simulink model "TIM_5_1_2"  (R2022b)
(part 3 of 4)

  Wire_16a (50) : M-S-Function  FunctionName=cisia_msfun  Parameters=Parameter1, Parameter2, Parameter3, resources, Parameter10, codeupdate, step_received, step_computed, dynamic_computed, step_sended, id_entity, id_project, id_type, name_type, color  mask(S-function:msfcn_unit_delay){Parameter1='Wire_16a', Parameter2=1, Parameter3='ORO', resources=|, Parameter10=off, codeupdate=off, step_received=|, step_computed=, dynamic_computed=, step_sended=|, id_entity=50, id_project=38, id_type=1, name_type=Optical_Wire, color=#99CCFF}
      mask resources=|
      | *** INPUT RESOURCES ***
      | NUM_INPUTS 4
      | TLC_CONN (20)
      | TLC_SERVICE (20)
      | CYBER_FAULT (10)
      | MECH_FAULT (1)
      |
      | *** STATE VARIABLES ***
      | NUM_VARIABLES 11
      | Operative_Level(NUMERIC)(1)(1)
      | TLC_services(NUMERIC_ARRAY)(20)(0  0  0  0  0  0  0  0  0  0  0  0  0  0  0  0  0  0  0  0)
      | Connection(NUMERIC_ARRAY)(20)(0  0  0  0  0  0  0  0  0  0  0  0  0  0  0  0  0  0  0  0)
      | Dos_attack(NUMERIC)(1)(0)
      | MITM_attack(NUMERIC)(1)(0)
      | Virus_Attack(NUMERIC)(1)(0)
      | Port_Scan_Attack(NUMERIC)(1)(0)
      | Cyber_Fault(NUMERIC_ARRAY)(10)(0  0  0  0  0  0  0  0  0  0)
      | Mechanical_Fault(NUMERIC)(1)(0)
      | Conn_Fault(NUMERIC)(1)(0)
      | TLC_revoke(NUMERIC_ARRAY)(20)(0  0  0  0  0  0  0  0  0  0  0  0  0  0  0  0  0  0  0  0)
      |
      | *** OUTPUT RESOURCES ***
      | NUM_OUTPUTS 4
      | TLC_CONN (20)
      | TLC_SERVICE (20)
      | CYBER_FAULT (10)
      | MECH_FAULT (1)
      mask step_received=|
      | Connection=max(Connection_init,TLC_CONN);
      | TLC_services=max(TLC_services_init,TLC_SERVICE);
      | TLC_services=mod(TLC_services,10);
      | TLC_revoke=floor(TLC_SERVICE/10);
      |
      | Cyber_Fault=CYBER_FAULT;
      |
      | Mechanical_Fault=max([Mechanical_Fault MECH_FAULT Mechanical_Fault_init]);
      |
      | %TLC_services=TLC_services.*(1-TLC_revoke);
      |
      | Operative_Level=1-Mechanical_Fault;
      mask step_sended=|
      | TLC_CONN=Connection*Operative_Level;
      | TLC_SERVICE=TLC_services*Operative_Level+TLC_revoke*10;
      |
      |
      | CYBER_FAULT=Cyber_Fault*Operative_Level;
      | MECH_FAULT=Mechanical_Fault;
      mask prompts: Parameter1 "entity name"; Parameter2 "sampling time"; Parameter3 "project"; resources "input resources and state variables"; Parameter10 "Bring state variables to output"; codeupdate "update code from mask"
      mask help: This is a level-2 MATLAB file S-function which demonstrates CISIA entity
      mask DialogControl Container1 Prompt: All parameters
      mask Display: image('Icons/Optical_Wire.png')
  Wire_17 (187) : M-S-Function  FunctionName=cisia_msfun  Parameters=Parameter1, Parameter2, Parameter3, resources, Parameter10, codeupdate, step_received, step_computed, dynamic_computed, step_sended, id_entity, id_project, id_type, name_type, color  mask(S-function:msfcn_unit_delay){Parameter1='Wire_17', Parameter2=1, Parameter3='ORO', resources=|, Parameter10=off, codeupdate=off, step_received=|, step_computed=, dynamic_computed=, step_sended=|, id_entity=187, id_project=38, id_type=1, name_type=Optical_Wire, color=#99CCFF}
      mask resources=|
      | *** INPUT RESOURCES ***
      | NUM_INPUTS 4
      | TLC_CONN (20)
      | TLC_SERVICE (20)
      | CYBER_FAULT (10)
      | MECH_FAULT (1)
      |
      | *** STATE VARIABLES ***
      | NUM_VARIABLES 11
      | Operative_Level(NUMERIC)(1)(1)
      | TLC_services(NUMERIC_ARRAY)(20)(0  0  0  0  0  0  0  0  0  0  0  0  0  0  0  0  0  0  0  0)
      | Connection(NUMERIC_ARRAY)(20)(0  0  0  0  0  0  0  0  0  0  0  0  0  0  0  0  0  0  0  0)
      | Dos_attack(NUMERIC)(1)(0)
      | MITM_attack(NUMERIC)(1)(0)
      | Virus_Attack(NUMERIC)(1)(0)
      | Port_Scan_Attack(NUMERIC)(1)(0)
      | Cyber_Fault(NUMERIC_ARRAY)(10)(0  0  0  0  0  0  0  0  0  0)
      | Mechanical_Fault(NUMERIC)(1)(0)
      | Conn_Fault(NUMERIC)(1)(0)
      | TLC_revoke(NUMERIC_ARRAY)(20)(0  0  0  0  0  0  0  0  0  0  0  0  0  0  0  0  0  0  0  0)
      |
      | *** OUTPUT RESOURCES ***
      | NUM_OUTPUTS 4
      | TLC_CONN (20)
      | TLC_SERVICE (20)
      | CYBER_FAULT (10)
      | MECH_FAULT (1)
      mask step_received=|
      | Connection=max(Connection_init,TLC_CONN);
      | TLC_services=max(TLC_services_init,TLC_SERVICE);
      | TLC_services=mod(TLC_services,10);
      | TLC_revoke=floor(TLC_SERVICE/10);
      |
      | Cyber_Fault=CYBER_FAULT;
      |
      | Mechanical_Fault=max([Mechanical_Fault MECH_FAULT Mechanical_Fault_init]);
      |
      | %TLC_services=TLC_services.*(1-TLC_revoke);
      |
      | Operative_Level=1-Mechanical_Fault;
      mask step_sended=|
      | TLC_CONN=Connection*Operative_Level;
      | TLC_SERVICE=TLC_services*Operative_Level+TLC_revoke*10;
      |
      |
      | CYBER_FAULT=Cyber_Fault*Operative_Level;
      | MECH_FAULT=Mechanical_Fault;
      mask prompts: Parameter1 "entity name"; Parameter2 "sampling time"; Parameter3 "project"; resources "input resources and state variables"; Parameter10 "Bring state variables to output"; codeupdate "update code from mask"
      mask help: This is a level-2 MATLAB file S-function which demonstrates CISIA entity
      mask DialogControl Container1 Prompt: All parameters
      mask Display: image('Icons/Optical_Wire.png')
  Wire_17b (188) : M-S-Function  FunctionName=cisia_msfun  Parameters=Parameter1, Parameter2, Parameter3, resources, Parameter10, codeupdate, step_received, step_computed, dynamic_computed, step_sended, id_entity, id_project, id_type, name_type, color  mask(S-function:msfcn_unit_delay){Parameter1='Wire_17b', Parameter2=1, Parameter3='ORO', resources=|, Parameter10=off, codeupdate=off, step_received=|, step_computed=, dynamic_computed=, step_sended=|, id_entity=188, id_project=38, id_type=1, name_type=Optical_Wire, color=#99CCFF}
      mask resources=|
      | *** INPUT RESOURCES ***
      | NUM_INPUTS 4
      | TLC_CONN (20)
      | TLC_SERVICE (20)
      | CYBER_FAULT (10)
      | MECH_FAULT (1)
      |
      | *** STATE VARIABLES ***
      | NUM_VARIABLES 11
      | Operative_Level(NUMERIC)(1)(1)
      | TLC_services(NUMERIC_ARRAY)(20)(0  0  0  0  0  0  0  0  0  0  0  0  0  0  0  0  0  0  0  0)
      | Connection(NUMERIC_ARRAY)(20)(0  0  0  0  0  0  0  0  0  0  0  0  0  0  0  0  0  0  0  0)
      | Dos_attack(NUMERIC)(1)(0)
      | MITM_attack(NUMERIC)(1)(0)
      | Virus_Attack(NUMERIC)(1)(0)
      | Port_Scan_Attack(NUMERIC)(1)(0)
      | Cyber_Fault(NUMERIC_ARRAY)(10)(0  0  0  0  0  0  0  0  0  0)
      | Mechanical_Fault(NUMERIC)(1)(0)
      | Conn_Fault(NUMERIC)(1)(0)
      | TLC_revoke(NUMERIC_ARRAY)(20)(0  0  0  0  0  0  0  0  0  0  0  0  0  0  0  0  0  0  0  0)
      |
      | *** OUTPUT RESOURCES ***
      | NUM_OUTPUTS 4
      | TLC_CONN (20)
      | TLC_SERVICE (20)
      | CYBER_FAULT (10)
      | MECH_FAULT (1)
      mask step_received=|
      | Connection=max(Connection_init,TLC_CONN);
      | TLC_services=max(TLC_services_init,TLC_SERVICE);
      | TLC_services=mod(TLC_services,10);
      | TLC_revoke=floor(TLC_SERVICE/10);
      |
      | Cyber_Fault=CYBER_FAULT;
      |
      | Mechanical_Fault=max([Mechanical_Fault MECH_FAULT Mechanical_Fault_init]);
      |
      | %TLC_services=TLC_services.*(1-TLC_revoke);
      |
      | Operative_Level=1-Mechanical_Fault;
      mask step_sended=|
      | TLC_CONN=Connection*Operative_Level;
      | TLC_SERVICE=TLC_services*Operative_Level+TLC_revoke*10;
      |
      |
      | CYBER_FAULT=Cyber_Fault*Operative_Level;
      | MECH_FAULT=Mechanical_Fault;
      mask prompts: Parameter1 "entity name"; Parameter2 "sampling time"; Parameter3 "project"; resources "input resources and state variables"; Parameter10 "Bring state variables to output"; codeupdate "update code from mask"
      mask help: This is a level-2 MATLAB file S-function which demonstrates CISIA entity
      mask DialogControl Container1 Prompt: All parameters
      mask Display: image('Icons/Optical_Wire.png')
  Wire_18 (190) : M-S-Function  FunctionName=cisia_msfun  Parameters=Parameter1, Parameter2, Parameter3, resources, Parameter10, codeupdate, step_received, step_computed, dynamic_computed, step_sended, id_entity, id_project, id_type, name_type, color  mask(S-function:msfcn_unit_delay){Parameter1='Wire_18', Parameter2=1, Parameter3='ORO', resources=|, Parameter10=off, codeupdate=off, step_received=|, step_computed=, dynamic_computed=, step_sended=|, id_entity=190, id_project=38, id_type=1, name_type=Optical_Wire, color=#99CCFF}
      mask resources=|
      | *** INPUT RESOURCES ***
      | NUM_INPUTS 4
      | TLC_CONN (20)
      | TLC_SERVICE (20)
      | CYBER_FAULT (10)
      | MECH_FAULT (1)
      |
      | *** STATE VARIABLES ***
      | NUM_VARIABLES 11
      | Operative_Level(NUMERIC)(1)(1)
      | TLC_services(NUMERIC_ARRAY)(20)(0  0  0  0  0  0  0  0  0  0  0  0  0  0  0  0  0  0  0  0)
      | Connection(NUMERIC_ARRAY)(20)(0  0  0  0  0  0  0  0  0  0  0  0  0  0  0  0  0  0  0  0)
      | Dos_attack(NUMERIC)(1)(0)
      | MITM_attack(NUMERIC)(1)(0)
      | Virus_Attack(NUMERIC)(1)(0)
      | Port_Scan_Attack(NUMERIC)(1)(0)
      | Cyber_Fault(NUMERIC_ARRAY)(10)(0  0  0  0  0  0  0  0  0  0)
      | Mechanical_Fault(NUMERIC)(1)(0)
      | Conn_Fault(NUMERIC)(1)(0)
      | TLC_revoke(NUMERIC_ARRAY)(20)(0  0  0  0  0  0  0  0  0  0  0  0  0  0  0  0  0  0  0  0)
      |
      | *** OUTPUT RESOURCES ***
      | NUM_OUTPUTS 4
      | TLC_CONN (20)
      | TLC_SERVICE (20)
      | CYBER_FAULT (10)
      | MECH_FAULT (1)
      mask step_received=|
      | Connection=max(Connection_init,TLC_CONN);
      | TLC_services=max(TLC_services_init,TLC_SERVICE);
      | TLC_services=mod(TLC_services,10);
      | TLC_revoke=floor(TLC_SERVICE/10);
      |
      | Cyber_Fault=CYBER_FAULT;
      |
      | Mechanical_Fault=max([Mechanical_Fault MECH_FAULT Mechanical_Fault_init]);
      |
      | %TLC_services=TLC_services.*(1-TLC_revoke);
      |
      | Operative_Level=1-Mechanical_Fault;
      mask step_sended=|
      | TLC_CONN=Connection*Operative_Level;
      | TLC_SERVICE=TLC_services*Operative_Level+TLC_revoke*10;
      |
      |
      | CYBER_FAULT=Cyber_Fault*Operative_Level;
      | MECH_FAULT=Mechanical_Fault;
      mask prompts: Parameter1 "entity name"; Parameter2 "sampling time"; Parameter3 "project"; resources "input resources and state variables"; Parameter10 "Bring state variables to output"; codeupdate "update code from mask"
      mask help: This is a level-2 MATLAB file S-function which demonstrates CISIA entity
      mask DialogControl Container1 Prompt: All parameters
      mask Display: image('Icons/Optical_Wire.png')
  Wire_18b (189) : M-S-Function  FunctionName=cisia_msfun  Parameters=Parameter1, Parameter2, Parameter3, resources, Parameter10, codeupdate, step_received, step_computed, dynamic_computed, step_sended, id_entity, id_project, id_type, name_type, color  mask(S-function:msfcn_unit_delay){Parameter1='Wire_18b', Parameter2=1, Parameter3='ORO', resources=|, Parameter10=off, codeupdate=off, step_received=|, step_computed=, dynamic_computed=, step_sended=|, id_entity=189, id_project=38, id_type=1, name_type=Optical_Wire, color=#99CCFF}
      mask resources=|
      | *** INPUT RESOURCES ***
      | NUM_INPUTS 4
      | TLC_CONN (20)
      | TLC_SERVICE (20)
      | CYBER_FAULT (10)
      | MECH_FAULT (1)
      |
      | *** STATE VARIABLES ***
      | NUM_VARIABLES 11
      | Operative_Level(NUMERIC)(1)(1)
      | TLC_services(NUMERIC_ARRAY)(20)(0  0  0  0  0  0  0  0  0  0  0  0  0  0  0  0  0  0  0  0)
      | Connection(NUMERIC_ARRAY)(20)(0  0  0  0  0  0  0  0  0  0  0  0  0  0  0  0  0  0  0  0)
      | Dos_attack(NUMERIC)(1)(0)
      | MITM_attack(NUMERIC)(1)(0)
      | Virus_Attack(NUMERIC)(1)(0)
      | Port_Scan_Attack(NUMERIC)(1)(0)
      | Cyber_Fault(NUMERIC_ARRAY)(10)(0  0  0  0  0  0  0  0  0  0)
      | Mechanical_Fault(NUMERIC)(1)(0)
      | Conn_Fault(NUMERIC)(1)(0)
      | TLC_revoke(NUMERIC_ARRAY)(20)(0  0  0  0  0  0  0  0  0  0  0  0  0  0  0  0  0  0  0  0)
      |
      | *** OUTPUT RESOURCES ***
      | NUM_OUTPUTS 4
      | TLC_CONN (20)
      | TLC_SERVICE (20)
      | CYBER_FAULT (10)
      | MECH_FAULT (1)
      mask step_received=|
      | Connection=max(Connection_init,TLC_CONN);
      | TLC_services=max(TLC_services_init,TLC_SERVICE);
      | TLC_services=mod(TLC_services,10);
      | TLC_revoke=floor(TLC_SERVICE/10);
      |
      | Cyber_Fault=CYBER_FAULT;
      |
      | Mechanical_Fault=max([Mechanical_Fault MECH_FAULT Mechanical_Fault_init]);
      |
      | %TLC_services=TLC_services.*(1-TLC_revoke);
      |
      | Operative_Level=1-Mechanical_Fault;
      mask step_sended=|
      | TLC_CONN=Connection*Operative_Level;
      | TLC_SERVICE=TLC_services*Operative_Level+TLC_revoke*10;
      |
      |
      | CYBER_FAULT=Cyber_Fault*Operative_Level;
      | MECH_FAULT=Mechanical_Fault;
      mask prompts: Parameter1 "entity name"; Parameter2 "sampling time"; Parameter3 "project"; resources "input resources and state variables"; Parameter10 "Bring state variables to output"; codeupdate "update code from mask"
      mask help: This is a level-2 MATLAB file S-function which demonstrates CISIA entity
      mask DialogControl Container1 Prompt: All parameters
      mask Display: image('Icons/Optical_Wire.png')
  Wire_19 (296) : M-S-Function  FunctionName=cisia_msfun  Parameters=Parameter1, Parameter2, Parameter3, resources, Parameter10, codeupdate, step_received, step_computed, dynamic_computed, step_sended, id_entity, id_project, id_type, name_type, color  mask(S-function:msfcn_unit_delay){Parameter1='Wire_19', Parameter2=1, Parameter3='ORO', resources=|, Parameter10=off, codeupdate=off, step_received=|, step_computed=, dynamic_computed=, step_sended=|, id_entity=296, id_project=38, id_type=1, name_type=Optical_Wire, color=#99CCFF}
      mask resources=|
      | *** INPUT RESOURCES ***
      | NUM_INPUTS 4
      | TLC_CONN (20)
      | TLC_SERVICE (20)
      | CYBER_FAULT (10)
      | MECH_FAULT (1)
      |
      | *** STATE VARIABLES ***
      | NUM_VARIABLES 11
      | Operative_Level(NUMERIC)(1)(1)
      | TLC_services(NUMERIC_ARRAY)(20)(0  0  0  0  0  0  0  0  0  0  0  0  0  0  0  0  0  0  0  0)
      | Connection(NUMERIC_ARRAY)(20)(0  0  0  0  0  0  0  0  0  0  0  0  0  0  0  0  0  0  0  0)
      | Dos_attack(NUMERIC)(1)(0)
      | MITM_attack(NUMERIC)(1)(0)
      | Virus_Attack(NUMERIC)(1)(0)
      | Port_Scan_Attack(NUMERIC)(1)(0)
      | Cyber_Fault(NUMERIC_ARRAY)(10)(0  0  0  0  0  0  0  0  0  0)
      | Mechanical_Fault(NUMERIC)(1)(0)
      | Conn_Fault(NUMERIC)(1)(0)
      | TLC_revoke(NUMERIC_ARRAY)(20)(0  0  0  0  0  0  0  0  0  0  0  0  0  0  0  0  0  0  0  0)
      |
      | *** OUTPUT RESOURCES ***
      | NUM_OUTPUTS 4
      | TLC_CONN (20)
      | TLC_SERVICE (20)
      | CYBER_FAULT (10)
      | MECH_FAULT (1)
      mask step_received=|
      | Connection=max(Connection_init,TLC_CONN);
      | TLC_services=max(TLC_services_init,TLC_SERVICE);
      | TLC_services=mod(TLC_services,10);
      | TLC_revoke=floor(TLC_SERVICE/10);
      |
      | Cyber_Fault=CYBER_FAULT;
      |
      | Mechanical_Fault=max([Mechanical_Fault MECH_FAULT Mechanical_Fault_init]);
      |
      | %TLC_services=TLC_services.*(1-TLC_revoke);
      |
      | Operative_Level=1-Mechanical_Fault;
      mask step_sended=|
      | TLC_CONN=Connection*Operative_Level;
      | TLC_SERVICE=TLC_services*Operative_Level+TLC_revoke*10;
      |
      |
      | CYBER_FAULT=Cyber_Fault*Operative_Level;
      | MECH_FAULT=Mechanical_Fault;
      mask prompts: Parameter1 "entity name"; Parameter2 "sampling time"; Parameter3 "project"; resources "input resources and state variables"; Parameter10 "Bring state variables to output"; codeupdate "update code from mask"
      mask help: This is a level-2 MATLAB file S-function which demonstrates CISIA entity
      mask DialogControl Container1 Prompt: All parameters
      mask Display: image('Icons/Optical_Wire.png')
  Wire_19b (297) : M-S-Function  FunctionName=cisia_msfun  Parameters=Parameter1, Parameter2, Parameter3, resources, Parameter10, codeupdate, step_received, step_computed, dynamic_computed, step_sended, id_entity, id_project, id_type, name_type, color  mask(S-function:msfcn_unit_delay){Parameter1='Wire_19b', Parameter2=1, Parameter3='ORO', resources=|, Parameter10=off, codeupdate=off, step_received=|, step_computed=, dynamic_computed=, step_sended=|, id_entity=297, id_project=38, id_type=1, name_type=Optical_Wire, color=#99CCFF}
      mask resources=|
      | *** INPUT RESOURCES ***
      | NUM_INPUTS 4
      | TLC_CONN (20)
      | TLC_SERVICE (20)
      | CYBER_FAULT (10)
      | MECH_FAULT (1)
      |
      | *** STATE VARIABLES ***
      | NUM_VARIABLES 11
      | Operative_Level(NUMERIC)(1)(1)
      | TLC_services(NUMERIC_ARRAY)(20)(0  0  0  0  0  0  0  0  0  0  0  0  0  0  0  0  0  0  0  0)
      | Connection(NUMERIC_ARRAY)(20)(0  0  0  0  0  0  0  0  0  0  0  0  0  0  0  0  0  0  0  0)
      | Dos_attack(NUMERIC)(1)(0)
      | MITM_attack(NUMERIC)(1)(0)
      | Virus_Attack(NUMERIC)(1)(0)
      | Port_Scan_Attack(NUMERIC)(1)(0)
      | Cyber_Fault(NUMERIC_ARRAY)(10)(0  0  0  0  0  0  0  0  0  0)
      | Mechanical_Fault(NUMERIC)(1)(0)
      | Conn_Fault(NUMERIC)(1)(0)
      | TLC_revoke(NUMERIC_ARRAY)(20)(0  0  0  0  0  0  0  0  0  0  0  0  0  0  0  0  0  0  0  0)
      |
      | *** OUTPUT RESOURCES ***
      | NUM_OUTPUTS 4
      | TLC_CONN (20)
      | TLC_SERVICE (20)
      | CYBER_FAULT (10)
      | MECH_FAULT (1)
      mask step_received=|
      | Connection=max(Connection_init,TLC_CONN);
      | TLC_services=max(TLC_services_init,TLC_SERVICE);
      | TLC_services=mod(TLC_services,10);
      | TLC_revoke=floor(TLC_SERVICE/10);
      |
      | Cyber_Fault=CYBER_FAULT;
      |
      | Mechanical_Fault=max([Mechanical_Fault MECH_FAULT Mechanical_Fault_init]);
      |
      | %TLC_services=TLC_services.*(1-TLC_revoke);
      |
      | Operative_Level=1-Mechanical_Fault;
      mask step_sended=|
      | TLC_CONN=Connection*Operative_Level;
      | TLC_SERVICE=TLC_services*Operative_Level+TLC_revoke*10;
      |
      |
      | CYBER_FAULT=Cyber_Fault*Operative_Level;
      | MECH_FAULT=Mechanical_Fault;
      mask prompts: Parameter1 "entity name"; Parameter2 "sampling time"; Parameter3 "project"; resources "input resources and state variables"; Parameter10 "Bring state variables to output"; codeupdate "update code from mask"
      mask help: This is a level-2 MATLAB file S-function which demonstrates CISIA entity
      mask DialogControl Container1 Prompt: All parameters
      mask Display: image('Icons/Optical_Wire.png')
  Wire_1b (96) : M-S-Function  FunctionName=cisia_msfun  Parameters=Parameter1, Parameter2, Parameter3, resources, Parameter10, codeupdate, step_received, step_computed, dynamic_computed, step_sended, id_entity, id_project, id_type, name_type, color  mask(S-function:msfcn_unit_delay){Parameter1='Wire_1b', Parameter2=1, Parameter3='ORO', resources=|, Parameter10=off, codeupdate=off, step_received=|, step_computed=, dynamic_computed=, step_sended=|, id_entity=96, id_project=38, id_type=1, name_type=Optical_Wire, color=#99CCFF}
      mask resources=|
      | *** INPUT RESOURCES ***
      | NUM_INPUTS 4
      | TLC_CONN (20)
      | TLC_SERVICE (20)
      | CYBER_FAULT (10)
      | MECH_FAULT (1)
      |
      | *** STATE VARIABLES ***
      | NUM_VARIABLES 11
      | Operative_Level(NUMERIC)(1)(1)
      | TLC_services(NUMERIC_ARRAY)(20)(0  0  0  0  0  0  0  0  0  0  0  0  0  0  0  0  0  0  0  0)
      | Connection(NUMERIC_ARRAY)(20)(0  0  0  0  0  0  0  0  0  0  0  0  0  0  0  0  0  0  0  0)
      | Dos_attack(NUMERIC)(1)(0)
      | MITM_attack(NUMERIC)(1)(0)
      | Virus_Attack(NUMERIC)(1)(0)
      | Port_Scan_Attack(NUMERIC)(1)(0)
      | Cyber_Fault(NUMERIC_ARRAY)(10)(0  0  0  0  0  0  0  0  0  0)
      | Mechanical_Fault(NUMERIC)(1)(0)
      | Conn_Fault(NUMERIC)(1)(0)
      | TLC_revoke(NUMERIC_ARRAY)(20)(0  0  0  0  0  0  0  0  0  0  0  0  0  0  0  0  0  0  0  0)
      |
      | *** OUTPUT RESOURCES ***
      | NUM_OUTPUTS 4
      | TLC_CONN (20)
      | TLC_SERVICE (20)
      | CYBER_FAULT (10)
      | MECH_FAULT (1)
      mask step_received=|
      | Connection=max(Connection_init,TLC_CONN);
      | TLC_services=max(TLC_services_init,TLC_SERVICE);
      | TLC_services=mod(TLC_services,10);
      | TLC_revoke=floor(TLC_SERVICE/10);
      |
      | Cyber_Fault=CYBER_FAULT;
      |
      | Mechanical_Fault=max([Mechanical_Fault MECH_FAULT Mechanical_Fault_init]);
      |
      | %TLC_services=TLC_services.*(1-TLC_revoke);
      |
      | Operative_Level=1-Mechanical_Fault;
      mask step_sended=|
      | TLC_CONN=Connection*Operative_Level;
      | TLC_SERVICE=TLC_services*Operative_Level+TLC_revoke*10;
      |
      |
      | CYBER_FAULT=Cyber_Fault*Operative_Level;
      | MECH_FAULT=Mechanical_Fault;
      mask prompts: Parameter1 "entity name"; Parameter2 "sampling time"; Parameter3 "project"; resources "input resources and state variables"; Parameter10 "Bring state variables to output"; codeupdate "update code from mask"
      mask help: This is a level-2 MATLAB file S-function which demonstrates CISIA entity
      mask DialogControl Container1 Prompt: All parameters
      mask Display: image('Icons/Optical_Wire.png')
  Wire_2 (2) : M-S-Function  FunctionName=cisia_msfun  Parameters=Parameter1, Parameter2, Parameter3, resources, Parameter10, codeupdate, step_received, step_computed, dynamic_computed, step_sended, id_entity, id_project, id_type, name_type, color  mask(S-function:msfcn_unit_delay){Parameter1='Wire_2', Parameter2=1, Parameter3='ORO', resources=|, Parameter10=off, codeupdate=off, step_received=|, step_computed=, dynamic_computed=, step_sended=|, id_entity=2, id_project=38, id_type=1, name_type=Optical_Wire, color=#99CCFF}
      mask resources=|
      | *** INPUT RESOURCES ***
      | NUM_INPUTS 4
      | TLC_CONN (20)
      | TLC_SERVICE (20)
      | CYBER_FAULT (10)
      | MECH_FAULT (1)
      |
      | *** STATE VARIABLES ***
      | NUM_VARIABLES 11
      | Operative_Level(NUMERIC)(1)(1)
      | TLC_services(NUMERIC_ARRAY)(20)(0  0  0  0  0  0  0  0  0  0  0  0  0  0  0  0  0  0  0  0)
      | Connection(NUMERIC_ARRAY)(20)(0  0  0  0  0  0  0  0  0  0  0  0  0  0  0  0  0  0  0  0)
      | Dos_attack(NUMERIC)(1)(0)
      | MITM_attack(NUMERIC)(1)(0)
      | Virus_Attack(NUMERIC)(1)(0)
      | Port_Scan_Attack(NUMERIC)(1)(0)
      | Cyber_Fault(NUMERIC_ARRAY)(10)(0  0  0  0  0  0  0  0  0  0)
      | Mechanical_Fault(NUMERIC)(1)(0)
      | Conn_Fault(NUMERIC)(1)(0)
      | TLC_revoke(NUMERIC_ARRAY)(20)(0  0  0  0  0  0  0  0  0  0  0  0  0  0  0  0  0  0  0  0)
      |
      | *** OUTPUT RESOURCES ***
      | NUM_OUTPUTS 4
      | TLC_CONN (20)
      | TLC_SERVICE (20)
      | CYBER_FAULT (10)
      | MECH_FAULT (1)
      mask step_received=|
      | Connection=max(Connection_init,TLC_CONN);
      | TLC_services=max(TLC_services_init,TLC_SERVICE);
      | TLC_services=mod(TLC_services,10);
      | TLC_revoke=floor(TLC_SERVICE/10);
      |
      | Cyber_Fault=CYBER_FAULT;
      |
      | Mechanical_Fault=max([Mechanical_Fault MECH_FAULT Mechanical_Fault_init]);
      |
      | %TLC_services=TLC_services.*(1-TLC_revoke);
      |
      | Operative_Level=1-Mechanical_Fault;
      mask step_sended=|
      | TLC_CONN=Connection*Operative_Level;
      | TLC_SERVICE=TLC_services*Operative_Level+TLC_revoke*10;
      |
      |
      | CYBER_FAULT=Cyber_Fault*Operative_Level;
      | MECH_FAULT=Mechanical_Fault;
      mask prompts: Parameter1 "entity name"; Parameter2 "sampling time"; Parameter3 "project"; resources "input resources and state variables"; Parameter10 "Bring state variables to output"; codeupdate "update code from mask"
      mask help: This is a level-2 MATLAB file S-function which demonstrates CISIA entity
      mask DialogControl Container1 Prompt: All parameters
      mask Display: image('Icons/Optical_Wire.png')
  Wire_2b (97) : M-S-Function  FunctionName=cisia_msfun  Parameters=Parameter1, Parameter2, Parameter3, resources, Parameter10, codeupdate, step_received, step_computed, dynamic_computed, step_sended, id_entity, id_project, id_type, name_type, color  mask(S-function:msfcn_unit_delay){Parameter1='Wire_2b', Parameter2=1, Parameter3='ORO', resources=|, Parameter10=off, codeupdate=off, step_received=|, step_computed=, dynamic_computed=, step_sended=|, id_entity=97, id_project=38, id_type=1, name_type=Optical_Wire, color=#99CCFF}
      mask resources=|
      | *** INPUT RESOURCES ***
      | NUM_INPUTS 4
      | TLC_CONN (20)
      | TLC_SERVICE (20)
      | CYBER_FAULT (10)
      | MECH_FAULT (1)
      |
      | *** STATE VARIABLES ***
      | NUM_VARIABLES 11
      | Operative_Level(NUMERIC)(1)(1)
      | TLC_services(NUMERIC_ARRAY)(20)(0  0  0  0  0  0  0  0  0  0  0  0  0  0  0  0  0  0  0  0)
      | Connection(NUMERIC_ARRAY)(20)(0  0  0  0  0  0  0  0  0  0  0  0  0  0  0  0  0  0  0  0)
      | Dos_attack(NUMERIC)(1)(0)
      | MITM_attack(NUMERIC)(1)(0)
      | Virus_Attack(NUMERIC)(1)(0)
      | Port_Scan_Attack(NUMERIC)(1)(0)
      | Cyber_Fault(NUMERIC_ARRAY)(10)(0  0  0  0  0  0  0  0  0  0)
      | Mechanical_Fault(NUMERIC)(1)(0)
      | Conn_Fault(NUMERIC)(1)(0)
      | TLC_revoke(NUMERIC_ARRAY)(20)(0  0  0  0  0  0  0  0  0  0  0  0  0  0  0  0  0  0  0  0)
      |
      | *** OUTPUT RESOURCES ***
      | NUM_OUTPUTS 4
      | TLC_CONN (20)
      | TLC_SERVICE (20)
      | CYBER_FAULT (10)
      | MECH_FAULT (1)
      mask step_received=|
      | Connection=max(Connection_init,TLC_CONN);
      | TLC_services=max(TLC_services_init,TLC_SERVICE);
      | TLC_services=mod(TLC_services,10);
      | TLC_revoke=floor(TLC_SERVICE/10);
      |
      | Cyber_Fault=CYBER_FAULT;
      |
      | Mechanical_Fault=max([Mechanical_Fault MECH_FAULT Mechanical_Fault_init]);
      |
      | %TLC_services=TLC_services.*(1-TLC_revoke);
      |
      | Operative_Level=1-Mechanical_Fault;
      mask step_sended=|
      | TLC_CONN=Connection*Operative_Level;
      | TLC_SERVICE=TLC_services*Operative_Level+TLC_revoke*10;
      |
      |
      | CYBER_FAULT=Cyber_Fault*Operative_Level;
      | MECH_FAULT=Mechanical_Fault;
      mask prompts: Parameter1 "entity name"; Parameter2 "sampling time"; Parameter3 "project"; resources "input resources and state variables"; Parameter10 "Bring state variables to output"; codeupdate "update code from mask"
      mask help: This is a level-2 MATLAB file S-function which demonstrates CISIA entity
      mask DialogControl Container1 Prompt: All parameters
      mask Display: image('Icons/Optical_Wire.png')
  Wire_3 (11) : M-S-Function  FunctionName=cisia_msfun  Parameters=Parameter1, Parameter2, Parameter3, resources, Parameter10, codeupdate, step_received, step_computed, dynamic_computed, step_sended, id_entity, id_project, id_type, name_type, color  mask(S-function:msfcn_unit_delay){Parameter1='Wire_3', Parameter2=1, Parameter3='ORO', resources=|, Parameter10=off, codeupdate=off, step_received=|, step_computed=, dynamic_computed=, step_sended=|, id_entity=11, id_project=38, id_type=1, name_type=Optical_Wire, color=#99CCFF}
      mask resources=|
      | *** INPUT RESOURCES ***
      | NUM_INPUTS 4
      | TLC_CONN (20)
      | TLC_SERVICE (20)
      | CYBER_FAULT (10)
      | MECH_FAULT (1)
      |
      | *** STATE VARIABLES ***
      | NUM_VARIABLES 11
      | Operative_Level(NUMERIC)(1)(1)
      | TLC_services(NUMERIC_ARRAY)(20)(0  0  0  0  0  0  0  0  0  0  0  0  0  0  0  0  0  0  0  0)
      | Connection(NUMERIC_ARRAY)(20)(0  0  0  0  0  0  0  0  0  0  0  0  0  0  0  0  0  0  0  0)
      | Dos_attack(NUMERIC)(1)(0)
      | MITM_attack(NUMERIC)(1)(0)
      | Virus_Attack(NUMERIC)(1)(0)
      | Port_Scan_Attack(NUMERIC)(1)(0)
      | Cyber_Fault(NUMERIC_ARRAY)(10)(0  0  0  0  0  0  0  0  0  0)
      | Mechanical_Fault(NUMERIC)(1)(0)
      | Conn_Fault(NUMERIC)(1)(0)
      | TLC_revoke(NUMERIC_ARRAY)(20)(0  0  0  0  0  0  0  0  0  0  0  0  0  0  0  0  0  0  0  0)
      |
      | *** OUTPUT RESOURCES ***
      | NUM_OUTPUTS 4
      | TLC_CONN (20)
      | TLC_SERVICE (20)
      | CYBER_FAULT (10)
      | MECH_FAULT (1)
      mask step_received=|
      | Connection=max(Connection_init,TLC_CONN);
      | TLC_services=max(TLC_services_init,TLC_SERVICE);
      | TLC_services=mod(TLC_services,10);
      | TLC_revoke=floor(TLC_SERVICE/10);
      |
      | Cyber_Fault=CYBER_FAULT;
      |
      | Mechanical_Fault=max([Mechanical_Fault MECH_FAULT Mechanical_Fault_init]);
      |
      | %TLC_services=TLC_services.*(1-TLC_revoke);
      |
      | Operative_Level=1-Mechanical_Fault;
      mask step_sended=|
      | TLC_CONN=Connection*Operative_Level;
      | TLC_SERVICE=TLC_services*Operative_Level+TLC_revoke*10;
      |
      |
      | CYBER_FAULT=Cyber_Fault*Operative_Level;
      | MECH_FAULT=Mechanical_Fault;
      mask prompts: Parameter1 "entity name"; Parameter2 "sampling time"; Parameter3 "project"; resources "input resources and state variables"; Parameter10 "Bring state variables to output"; codeupdate "update code from mask"
      mask help: This is a level-2 MATLAB file S-function which demonstrates CISIA entity
      mask DialogControl Container1 Prompt: All parameters
      mask Display: image('Icons/Optical_Wire.png')
  Wire_3b (14) : M-S-Function  FunctionName=cisia_msfun  Parameters=Parameter1, Parameter2, Parameter3, resources, Parameter10, codeupdate, step_received, step_computed, dynamic_computed, step_sended, id_entity, id_project, id_type, name_type, color  mask(S-function:msfcn_unit_delay){Parameter1='Wire_3b', Parameter2=1, Parameter3='ORO', resources=|, Parameter10=off, codeupdate=off, step_received=|, step_computed=, dynamic_computed=, step_sended=|, id_entity=14, id_project=38, id_type=1, name_type=Optical_Wire, color=#99CCFF}
      mask resources=|
      | *** INPUT RESOURCES ***
      | NUM_INPUTS 4
      | TLC_CONN (20)
      | TLC_SERVICE (20)
      | CYBER_FAULT (10)
      | MECH_FAULT (1)
      |
      | *** STATE VARIABLES ***
      | NUM_VARIABLES 11
      | Operative_Level(NUMERIC)(1)(1)
      | TLC_services(NUMERIC_ARRAY)(20)(0  0  0  0  0  0  0  0  0  0  0  0  0  0  0  0  0  0  0  0)
      | Connection(NUMERIC_ARRAY)(20)(0  0  0  0  0  0  0  0  0  0  0  0  0  0  0  0  0  0  0  0)
      | Dos_attack(NUMERIC)(1)(0)
      | MITM_attack(NUMERIC)(1)(0)
      | Virus_Attack(NUMERIC)(1)(0)
      | Port_Scan_Attack(NUMERIC)(1)(0)
      | Cyber_Fault(NUMERIC_ARRAY)(10)(0  0  0  0  0  0  0  0  0  0)
      | Mechanical_Fault(NUMERIC)(1)(0)
      | Conn_Fault(NUMERIC)(1)(0)
      | TLC_revoke(NUMERIC_ARRAY)(20)(0  0  0  0  0  0  0  0  0  0  0  0  0  0  0  0  0  0  0  0)
      |
      | *** OUTPUT RESOURCES ***
      | NUM_OUTPUTS 4
      | TLC_CONN (20)
      | TLC_SERVICE (20)
      | CYBER_FAULT (10)
      | MECH_FAULT (1)
      mask step_received=|
      | Connection=max(Connection_init,TLC_CONN);
      | TLC_services=max(TLC_services_init,TLC_SERVICE);
      | TLC_services=mod(TLC_services,10);
      | TLC_revoke=floor(TLC_SERVICE/10);
      |
      | Cyber_Fault=CYBER_FAULT;
      |
      | Mechanical_Fault=max([Mechanical_Fault MECH_FAULT Mechanical_Fault_init]);
      |
      | %TLC_services=TLC_services.*(1-TLC_revoke);
      |
      | Operative_Level=1-Mechanical_Fault;
      mask step_sended=|
      | TLC_CONN=Connection*Operative_Level;
      | TLC_SERVICE=TLC_services*Operative_Level+TLC_revoke*10;
      |
      |
      | CYBER_FAULT=Cyber_Fault*Operative_Level;
      | MECH_FAULT=Mechanical_Fault;
      mask prompts: Parameter1 "entity name"; Parameter2 "sampling time"; Parameter3 "project"; resources "input resources and state variables"; Parameter10 "Bring state variables to output"; codeupdate "update code from mask"
      mask help: This is a level-2 MATLAB file S-function which demonstrates CISIA entity
      mask DialogControl Container1 Prompt: All parameters
      mask Display: image('Icons/Optical_Wire.png')
  Wire_4 (12) : M-S-Function  FunctionName=cisia_msfun  Parameters=Parameter1, Parameter2, Parameter3, resources, Parameter10, codeupdate, step_received, step_computed, dynamic_computed, step_sended, id_entity, id_project, id_type, name_type, color  mask(S-function:msfcn_unit_delay){Parameter1='Wire_4', Parameter2=1, Parameter3='ORO', resources=|, Parameter10=off, codeupdate=off, step_received=|, step_computed=, dynamic_computed=, step_sended=|, id_entity=12, id_project=38, id_type=1, name_type=Optical_Wire, color=#99CCFF}
      mask resources=|
      | *** INPUT RESOURCES ***
      | NUM_INPUTS 4
      | TLC_CONN (20)
      | TLC_SERVICE (20)
      | CYBER_FAULT (10)
      | MECH_FAULT (1)
      |
      | *** STATE VARIABLES ***
      | NUM_VARIABLES 11
      | Operative_Level(NUMERIC)(1)(1)
      | TLC_services(NUMERIC_ARRAY)(20)(0  0  0  0  0  0  0  0  0  0  0  0  0  0  0  0  0  0  0  0)
      | Connection(NUMERIC_ARRAY)(20)(0  0  0  0  0  0  0  0  0  0  0  0  0  0  0  0  0  0  0  0)
      | Dos_attack(NUMERIC)(1)(0)
      | MITM_attack(NUMERIC)(1)(0)
      | Virus_Attack(NUMERIC)(1)(0)
      | Port_Scan_Attack(NUMERIC)(1)(0)
      | Cyber_Fault(NUMERIC_ARRAY)(10)(0  0  0  0  0  0  0  0  0  0)
      | Mechanical_Fault(NUMERIC)(1)(0)
      | Conn_Fault(NUMERIC)(1)(0)
      | TLC_revoke(NUMERIC_ARRAY)(20)(0  0  0  0  0  0  0  0  0  0  0  0  0  0  0  0  0  0  0  0)
      |
      | *** OUTPUT RESOURCES ***
      | NUM_OUTPUTS 4
      | TLC_CONN (20)
      | TLC_SERVICE (20)
      | CYBER_FAULT (10)
      | MECH_FAULT (1)
      mask step_received=|
      | Connection=max(Connection_init,TLC_CONN);
      | TLC_services=max(TLC_services_init,TLC_SERVICE);
      | TLC_services=mod(TLC_services,10);
      | TLC_revoke=floor(TLC_SERVICE/10);
      |
      | Cyber_Fault=CYBER_FAULT;
      |
      | Mechanical_Fault=max([Mechanical_Fault MECH_FAULT Mechanical_Fault_init]);
      |
      | %TLC_services=TLC_services.*(1-TLC_revoke);
      |
      | Operative_Level=1-Mechanical_Fault;
      mask step_sended=|
      | TLC_CONN=Connection*Operative_Level;
      | TLC_SERVICE=TLC_services*Operative_Level+TLC_revoke*10;
      |
      |
      | CYBER_FAULT=Cyber_Fault*Operative_Level;
      | MECH_FAULT=Mechanical_Fault;
      mask prompts: Parameter1 "entity name"; Parameter2 "sampling time"; Parameter3 "project"; resources "input resources and state variables"; Parameter10 "Bring state variables to output"; codeupdate "update code from mask"
      mask help: This is a level-2 MATLAB file S-function which demonstrates CISIA entity
      mask DialogControl Container1 Prompt: All parameters
      mask Display: image('Icons/Optical_Wire.png')
  Wire_4b (13) : M-S-Function  FunctionName=cisia_msfun  Parameters=Parameter1, Parameter2, Parameter3, resources, Parameter10, codeupdate, step_received, step_computed, dynamic_computed, step_sended, id_entity, id_project, id_type, name_type, color  mask(S-function:msfcn_unit_delay){Parameter1='Wire_4b', Parameter2=1, Parameter3='ORO', resources=|, Parameter10=off, codeupdate=off, step_received=|, step_computed=, dynamic_computed=, step_sended=|, id_entity=13, id_project=38, id_type=1, name_type=Optical_Wire, color=#99CCFF}
      mask resources=|
      | *** INPUT RESOURCES ***
      | NUM_INPUTS 4
      | TLC_CONN (20)
      | TLC_SERVICE (20)
      | CYBER_FAULT (10)
      | MECH_FAULT (1)
      |
      | *** STATE VARIABLES ***
      | NUM_VARIABLES 11
      | Operative_Level(NUMERIC)(1)(1)
      | TLC_services(NUMERIC_ARRAY)(20)(0  0  0  0  0  0  0  0  0  0  0  0  0  0  0  0  0  0  0  0)
      | Connection(NUMERIC_ARRAY)(20)(0  0  0  0  0  0  0  0  0  0  0  0  0  0  0  0  0  0  0  0)
      | Dos_attack(NUMERIC)(1)(0)
      | MITM_attack(NUMERIC)(1)(0)
      | Virus_Attack(NUMERIC)(1)(0)
      | Port_Scan_Attack(NUMERIC)(1)(0)
      | Cyber_Fault(NUMERIC_ARRAY)(10)(0  0  0  0  0  0  0  0  0  0)
      | Mechanical_Fault(NUMERIC)(1)(0)
      | Conn_Fault(NUMERIC)(1)(0)
      | TLC_revoke(NUMERIC_ARRAY)(20)(0  0  0  0  0  0  0  0  0  0  0  0  0  0  0  0  0  0  0  0)
      |
      | *** OUTPUT RESOURCES ***
      | NUM_OUTPUTS 4
      | TLC_CONN (20)
      | TLC_SERVICE (20)
      | CYBER_FAULT (10)
      | MECH_FAULT (1)
      mask step_received=|
      | Connection=max(Connection_init,TLC_CONN);
      | TLC_services=max(TLC_services_init,TLC_SERVICE);
      | TLC_services=mod(TLC_services,10);
      | TLC_revoke=floor(TLC_SERVICE/10);
      |
      | Cyber_Fault=CYBER_FAULT;
      |
      | Mechanical_Fault=max([Mechanical_Fault MECH_FAULT Mechanical_Fault_init]);
      |
      | %TLC_services=TLC_services.*(1-TLC_revoke);
      |
      | Operative_Level=1-Mechanical_Fault;
      mask step_sended=|
      | TLC_CONN=Connection*Operative_Level;
      | TLC_SERVICE=TLC_services*Operative_Level+TLC_revoke*10;
      |
      |
      | CYBER_FAULT=Cyber_Fault*Operative_Level;
      | MECH_FAULT=Mechanical_Fault;
      mask prompts: Parameter1 "entity name"; Parameter2 "sampling time"; Parameter3 "project"; resources "input resources and state variables"; Parameter10 "Bring state variables to output"; codeupdate "update code from mask"
      mask help: This is a level-2 MATLAB file S-function which demonstrates CISIA entity
      mask DialogControl Container1 Prompt: All parameters
      mask Display: image('Icons/Optical_Wire.png')
  Wire_5 (15) : M-S-Function  FunctionName=cisia_msfun  Parameters=Parameter1, Parameter2, Parameter3, resources, Parameter10, codeupdate, step_received, step_computed, dynamic_computed, step_sended, id_entity, id_project, id_type, name_type, color  mask(S-function:msfcn_unit_delay){Parameter1='Wire_5', Parameter2=1, Parameter3='ORO', resources=|, Parameter10=off, codeupdate=off, step_received=|, step_computed=, dynamic_computed=, step_sended=|, id_entity=15, id_project=38, id_type=1, name_type=Optical_Wire, color=#99CCFF}
      mask resources=|
      | *** INPUT RESOURCES ***
      | NUM_INPUTS 4
      | TLC_CONN (20)
      | TLC_SERVICE (20)
      | CYBER_FAULT (10)
      | MECH_FAULT (1)
      |
      | *** STATE VARIABLES ***
      | NUM_VARIABLES 11
      | Operative_Level(NUMERIC)(1)(1)
      | TLC_services(NUMERIC_ARRAY)(20)(0  0  0  0  0  0  0  0  0  0  0  0  0  0  0  0  0  0  0  0)
      | Connection(NUMERIC_ARRAY)(20)(0  0  0  0  0  0  0  0  0  0  0  0  0  0  0  0  0  0  0  0)
      | Dos_attack(NUMERIC)(1)(0)
      | MITM_attack(NUMERIC)(1)(0)
      | Virus_Attack(NUMERIC)(1)(0)
      | Port_Scan_Attack(NUMERIC)(1)(0)
      | Cyber_Fault(NUMERIC_ARRAY)(10)(0  0  0  0  0  0  0  0  0  0)
      | Mechanical_Fault(NUMERIC)(1)(0)
      | Conn_Fault(NUMERIC)(1)(0)
      | TLC_revoke(NUMERIC_ARRAY)(20)(0  0  0  0  0  0  0  0  0  0  0  0  0  0  0  0  0  0  0  0)
      |
      | *** OUTPUT RESOURCES ***
      | NUM_OUTPUTS 4
      | TLC_CONN (20)
      | TLC_SERVICE (20)
      | CYBER_FAULT (10)
      | MECH_FAULT (1)
      mask step_received=|
      | Connection=max(Connection_init,TLC_CONN);
      | TLC_services=max(TLC_services_init,TLC_SERVICE);
      | TLC_services=mod(TLC_services,10);
      | TLC_revoke=floor(TLC_SERVICE/10);
      |
      | Cyber_Fault=CYBER_FAULT;
      |
      | Mechanical_Fault=max([Mechanical_Fault MECH_FAULT Mechanical_Fault_init]);
      |
      | %TLC_services=TLC_services.*(1-TLC_revoke);
      |
      | Operative_Level=1-Mechanical_Fault;
      mask step_sended=|
      | TLC_CONN=Connection*Operative_Level;
      | TLC_SERVICE=TLC_services*Operative_Level+TLC_revoke*10;
      |
      |
      | CYBER_FAULT=Cyber_Fault*Operative_Level;
      | MECH_FAULT=Mechanical_Fault;
      mask prompts: Parameter1 "entity name"; Parameter2 "sampling time"; Parameter3 "project"; resources "input resources and state variables"; Parameter10 "Bring state variables to output"; codeupdate "update code from mask"
      mask help: This is a level-2 MATLAB file S-function which demonstrates CISIA entity
      mask DialogControl Container1 Prompt: All parameters
      mask Display: image('Icons/Optical_Wire.png')
  Wire_5b (16) : M-S-Function  FunctionName=cisia_msfun  Parameters=Parameter1, Parameter2, Parameter3, resources, Parameter10, codeupdate, step_received, step_computed, dynamic_computed, step_sended, id_entity, id_project, id_type, name_type, color  mask(S-function:msfcn_unit_delay){Parameter1='Wire_5b', Parameter2=1, Parameter3='ORO', resources=|, Parameter10=off, codeupdate=off, step_received=|, step_computed=, dynamic_computed=, step_sended=|, id_entity=16, id_project=38, id_type=1, name_type=Optical_Wire, color=#99CCFF}
      mask resources=|
      | *** INPUT RESOURCES ***
      | NUM_INPUTS 4
      | TLC_CONN (20)
      | TLC_SERVICE (20)
      | CYBER_FAULT (10)
      | MECH_FAULT (1)
      |
      | *** STATE VARIABLES ***
      | NUM_VARIABLES 11
      | Operative_Level(NUMERIC)(1)(1)
      | TLC_services(NUMERIC_ARRAY)(20)(0  0  0  0  0  0  0  0  0  0  0  0  0  0  0  0  0  0  0  0)
      | Connection(NUMERIC_ARRAY)(20)(0  0  0  0  0  0  0  0  0  0  0  0  0  0  0  0  0  0  0  0)
      | Dos_attack(NUMERIC)(1)(0)
      | MITM_attack(NUMERIC)(1)(0)
      | Virus_Attack(NUMERIC)(1)(0)
      | Port_Scan_Attack(NUMERIC)(1)(0)
      | Cyber_Fault(NUMERIC_ARRAY)(10)(0  0  0  0  0  0  0  0  0  0)
      | Mechanical_Fault(NUMERIC)(1)(0)
      | Conn_Fault(NUMERIC)(1)(0)
      | TLC_revoke(NUMERIC_ARRAY)(20)(0  0  0  0  0  0  0  0  0  0  0  0  0  0  0  0  0  0  0  0)
      |
      | *** OUTPUT RESOURCES ***
      | NUM_OUTPUTS 4
      | TLC_CONN (20)
      | TLC_SERVICE (20)
      | CYBER_FAULT (10)
      | MECH_FAULT (1)
      mask step_received=|
      | Connection=max(Connection_init,TLC_CONN);
      | TLC_services=max(TLC_services_init,TLC_SERVICE);
      | TLC_services=mod(TLC_services,10);
      | TLC_revoke=floor(TLC_SERVICE/10);
      |
      | Cyber_Fault=CYBER_FAULT;
      |
      | Mechanical_Fault=max([Mechanical_Fault MECH_FAULT Mechanical_Fault_init]);
      |
      | %TLC_services=TLC_services.*(1-TLC_revoke);
      |
      | Operative_Level=1-Mechanical_Fault;
      mask step_sended=|
      | TLC_CONN=Connection*Operative_Level;
      | TLC_SERVICE=TLC_services*Operative_Level+TLC_revoke*10;
      |
      |
      | CYBER_FAULT=Cyber_Fault*Operative_Level;
      | MECH_FAULT=Mechanical_Fault;
      mask prompts: Parameter1 "entity name"; Parameter2 "sampling time"; Parameter3 "project"; resources "input resources and state variables"; Parameter10 "Bring state variables to output"; codeupdate "update code from mask"
      mask help: This is a level-2 MATLAB file S-function which demonstrates CISIA entity
      mask DialogControl Container1 Prompt: All parameters
      mask Display: image('Icons/Optical_Wire.png')
  Wire_6 (17) : M-S-Function  FunctionName=cisia_msfun  Parameters=Parameter1, Parameter2, Parameter3, resources, Parameter10, codeupdate, step_received, step_computed, dynamic_computed, step_sended, id_entity, id_project, id_type, name_type, color  mask(S-function:msfcn_unit_delay){Parameter1='Wire_6', Parameter2=1, Parameter3='ORO', resources=|, Parameter10=off, codeupdate=off, step_received=|, step_computed=, dynamic_computed=, step_sended=|, id_entity=17, id_project=38, id_type=1, name_type=Optical_Wire, color=#99CCFF}
      mask resources=|
      | *** INPUT RESOURCES ***
      | NUM_INPUTS 4
      | TLC_CONN (20)
      | TLC_SERVICE (20)
      | CYBER_FAULT (10)
      | MECH_FAULT (1)
      |
      | *** STATE VARIABLES ***
      | NUM_VARIABLES 11
      | Operative_Level(NUMERIC)(1)(1)
      | TLC_services(NUMERIC_ARRAY)(20)(0  0  0  0  0  0  0  0  0  0  0  0  0  0  0  0  0  0  0  0)
      | Connection(NUMERIC_ARRAY)(20)(0  0  0  0  0  0  0  0  0  0  0  0  0  0  0  0  0  0  0  0)
      | Dos_attack(NUMERIC)(1)(0)
      | MITM_attack(NUMERIC)(1)(0)
      | Virus_Attack(NUMERIC)(1)(0)
      | Port_Scan_Attack(NUMERIC)(1)(0)
      | Cyber_Fault(NUMERIC_ARRAY)(10)(0  0  0  0  0  0  0  0  0  0)
      | Mechanical_Fault(NUMERIC)(1)(0)
      | Conn_Fault(NUMERIC)(1)(0)
      | TLC_revoke(NUMERIC_ARRAY)(20)(0  0  0  0  0  0  0  0  0  0  0  0  0  0  0  0  0  0  0  0)
      |
      | *** OUTPUT RESOURCES ***
      | NUM_OUTPUTS 4
      | TLC_CONN (20)
      | TLC_SERVICE (20)
      | CYBER_FAULT (10)
      | MECH_FAULT (1)
      mask step_received=|
      | Connection=max(Connection_init,TLC_CONN);
      | TLC_services=max(TLC_services_init,TLC_SERVICE);
      | TLC_services=mod(TLC_services,10);
      | TLC_revoke=floor(TLC_SERVICE/10);
      |
      | Cyber_Fault=CYBER_FAULT;
      |
      | Mechanical_Fault=max([Mechanical_Fault MECH_FAULT Mechanical_Fault_init]);
      |
      | %TLC_services=TLC_services.*(1-TLC_revoke);
      |
      | Operative_Level=1-Mechanical_Fault;
      mask step_sended=|
      | TLC_CONN=Connection*Operative_Level;
      | TLC_SERVICE=TLC_services*Operative_Level+TLC_revoke*10;
      |
      |
      | CYBER_FAULT=Cyber_Fault*Operative_Level;
      | MECH_FAULT=Mechanical_Fault;
      mask prompts: Parameter1 "entity name"; Parameter2 "sampling time"; Parameter3 "project"; resources "input resources and state variables"; Parameter10 "Bring state variables to output"; codeupdate "update code from mask"
      mask help: This is a level-2 MATLAB file S-function which demonstrates CISIA entity
      mask DialogControl Container1 Prompt: All parameters
      mask Display: image('Icons/Optical_Wire.png')
  Wire_6b (18) : M-S-Function  FunctionName=cisia_msfun  Parameters=Parameter1, Parameter2, Parameter3, resources, Parameter10, codeupdate, step_received, step_computed, dynamic_computed, step_sended, id_entity, id_project, id_type, name_type, color  mask(S-function:msfcn_unit_delay){Parameter1='Wire_6b', Parameter2=1, Parameter3='ORO', resources=|, Parameter10=off, codeupdate=off, step_received=|, step_computed=, dynamic_computed=, step_sended=|, id_entity=18, id_project=38, id_type=1, name_type=Optical_Wire, color=#99CCFF}
      mask resources=|
      | *** INPUT RESOURCES ***
      | NUM_INPUTS 4
      | TLC_CONN (20)
      | TLC_SERVICE (20)
      | CYBER_FAULT (10)
      | MECH_FAULT (1)
      |
      | *** STATE VARIABLES ***
      | NUM_VARIABLES 11
      | Operative_Level(NUMERIC)(1)(1)
      | TLC_services(NUMERIC_ARRAY)(20)(0  0  0  0  0  0  0  0  0  0  0  0  0  0  0  0  0  0  0  0)
      | Connection(NUMERIC_ARRAY)(20)(0  0  0  0  0  0  0  0  0  0  0  0  0  0  0  0  0  0  0  0)
      | Dos_attack(NUMERIC)(1)(0)
      | MITM_attack(NUMERIC)(1)(0)
      | Virus_Attack(NUMERIC)(1)(0)
      | Port_Scan_Attack(NUMERIC)(1)(0)
      | Cyber_Fault(NUMERIC_ARRAY)(10)(0  0  0  0  0  0  0  0  0  0)
      | Mechanical_Fault(NUMERIC)(1)(0)
      | Conn_Fault(NUMERIC)(1)(0)
      | TLC_revoke(NUMERIC_ARRAY)(20)(0  0  0  0  0  0  0  0  0  0  0  0  0  0  0  0  0  0  0  0)
      |
      | *** OUTPUT RESOURCES ***
      | NUM_OUTPUTS 4
      | TLC_CONN (20)
      | TLC_SERVICE (20)
      | CYBER_FAULT (10)
      | MECH_FAULT (1)
      mask step_received=|
      | Connection=max(Connection_init,TLC_CONN);
      | TLC_services=max(TLC_services_init,TLC_SERVICE);
      | TLC_services=mod(TLC_services,10);
      | TLC_revoke=floor(TLC_SERVICE/10);
      |
      | Cyber_Fault=CYBER_FAULT;
      |
      | Mechanical_Fault=max([Mechanical_Fault MECH_FAULT Mechanical_Fault_init]);
      |
      | %TLC_services=TLC_services.*(1-TLC_revoke);
      |
      | Operative_Level=1-Mechanical_Fault;
      mask step_sended=|
      | TLC_CONN=Connection*Operative_Level;
      | TLC_SERVICE=TLC_services*Operative_Level+TLC_revoke*10;
      |
      |
      | CYBER_FAULT=Cyber_Fault*Operative_Level;
      | MECH_FAULT=Mechanical_Fault;
      mask prompts: Parameter1 "entity name"; Parameter2 "sampling time"; Parameter3 "project"; resources "input resources and state variables"; Parameter10 "Bring state variables to output"; codeupdate "update code from mask"
      mask help: This is a level-2 MATLAB file S-function which demonstrates CISIA entity
      mask DialogControl Container1 Prompt: All parameters
      mask Display: image('Icons/Optical_Wire.png')
  Wire_7 (19) : M-S-Function  FunctionName=cisia_msfun  Parameters=Parameter1, Parameter2, Parameter3, resources, Parameter10, codeupdate, step_received, step_computed, dynamic_computed, step_sended, id_entity, id_project, id_type, name_type, color  mask(S-function:msfcn_unit_delay){Parameter1='Wire_7', Parameter2=1, Parameter3='ORO', resources=|, Parameter10=off, codeupdate=off, step_received=|, step_computed=, dynamic_computed=, step_sended=|, id_entity=19, id_project=38, id_type=1, name_type=Optical_Wire, color=#99CCFF}
      mask resources=|
      | *** INPUT RESOURCES ***
      | NUM_INPUTS 4
      | TLC_CONN (20)
      | TLC_SERVICE (20)
      | CYBER_FAULT (10)
      | MECH_FAULT (1)
      |
      | *** STATE VARIABLES ***
      | NUM_VARIABLES 11
      | Operative_Level(NUMERIC)(1)(1)
      | TLC_services(NUMERIC_ARRAY)(20)(0  0  0  0  0  0  0  0  0  0  0  0  0  0  0  0  0  0  0  0)
      | Connection(NUMERIC_ARRAY)(20)(0  0  0  0  0  0  0  0  0  0  0  0  0  0  0  0  0  0  0  0)
      | Dos_attack(NUMERIC)(1)(0)
      | MITM_attack(NUMERIC)(1)(0)
      | Virus_Attack(NUMERIC)(1)(0)
      | Port_Scan_Attack(NUMERIC)(1)(0)
      | Cyber_Fault(NUMERIC_ARRAY)(10)(0  0  0  0  0  0  0  0  0  0)
      | Mechanical_Fault(NUMERIC)(1)(0)
      | Conn_Fault(NUMERIC)(1)(0)
      | TLC_revoke(NUMERIC_ARRAY)(20)(0  0  0  0  0  0  0  0  0  0  0  0  0  0  0  0  0  0  0  0)
      |
      | *** OUTPUT RESOURCES ***
      | NUM_OUTPUTS 4
      | TLC_CONN (20)
      | TLC_SERVICE (20)
      | CYBER_FAULT (10)
      | MECH_FAULT (1)
      mask step_received=|
      | Connection=max(Connection_init,TLC_CONN);
      | TLC_services=max(TLC_services_init,TLC_SERVICE);
      | TLC_services=mod(TLC_services,10);
      | TLC_revoke=floor(TLC_SERVICE/10);
      |
      | Cyber_Fault=CYBER_FAULT;
      |
      | Mechanical_Fault=max([Mechanical_Fault MECH_FAULT Mechanical_Fault_init]);
      |
      | %TLC_services=TLC_services.*(1-TLC_revoke);
      |
      | Operative_Level=1-Mechanical_Fault;
      mask step_sended=|
      | TLC_CONN=Connection*Operative_Level;
      | TLC_SERVICE=TLC_services*Operative_Level+TLC_revoke*10;
      |
      |
      | CYBER_FAULT=Cyber_Fault*Operative_Level;
      | MECH_FAULT=Mechanical_Fault;
      mask prompts: Parameter1 "entity name"; Parameter2 "sampling time"; Parameter3 "project"; resources "input resources and state variables"; Parameter10 "Bring state variables to output"; codeupdate "update code from mask"
      mask help: This is a level-2 MATLAB file S-function which demonstrates CISIA entity
      mask DialogControl Container1 Prompt: All parameters
      mask Display: image('Icons/Optical_Wire.png')
  Wire_7b (20) : M-S-Function  FunctionName=cisia_msfun  Parameters=Parameter1, Parameter2, Parameter3, resources, Parameter10, codeupdate, step_received, step_computed, dynamic_computed, step_sended, id_entity, id_project, id_type, name_type, color  mask(S-function:msfcn_unit_delay){Parameter1='Wire_7b', Parameter2=1, Parameter3='ORO', resources=|, Parameter10=off, codeupdate=off, step_received=|, step_computed=, dynamic_computed=, step_sended=|, id_entity=20, id_project=38, id_type=1, name_type=Optical_Wire, color=#99CCFF}
      mask resources=|
      | *** INPUT RESOURCES ***
      | NUM_INPUTS 4
      | TLC_CONN (20)
      | TLC_SERVICE (20)
      | CYBER_FAULT (10)
      | MECH_FAULT (1)
      |
      | *** STATE VARIABLES ***
      | NUM_VARIABLES 11
      | Operative_Level(NUMERIC)(1)(1)
      | TLC_services(NUMERIC_ARRAY)(20)(0  0  0  0  0  0  0  0  0  0  0  0  0  0  0  0  0  0  0  0)
      | Connection(NUMERIC_ARRAY)(20)(0  0  0  0  0  0  0  0  0  0  0  0  0  0  0  0  0  0  0  0)
      | Dos_attack(NUMERIC)(1)(0)
      | MITM_attack(NUMERIC)(1)(0)
      | Virus_Attack(NUMERIC)(1)(0)
      | Port_Scan_Attack(NUMERIC)(1)(0)
      | Cyber_Fault(NUMERIC_ARRAY)(10)(0  0  0  0  0  0  0  0  0  0)
      | Mechanical_Fault(NUMERIC)(1)(0)
      | Conn_Fault(NUMERIC)(1)(0)
      | TLC_revoke(NUMERIC_ARRAY)(20)(0  0  0  0  0  0  0  0  0  0  0  0  0  0  0  0  0  0  0  0)
      |
      | *** OUTPUT RESOURCES ***
      | NUM_OUTPUTS 4
      | TLC_CONN (20)
      | TLC_SERVICE (20)
      | CYBER_FAULT (10)
      | MECH_FAULT (1)
      mask step_received=|
      | Connection=max(Connection_init,TLC_CONN);
      | TLC_services=max(TLC_services_init,TLC_SERVICE);
      | TLC_services=mod(TLC_services,10);
      | TLC_revoke=floor(TLC_SERVICE/10);
      |
      | Cyber_Fault=CYBER_FAULT;
      |
      | Mechanical_Fault=max([Mechanical_Fault MECH_FAULT Mechanical_Fault_init]);
      |
      | %TLC_services=TLC_services.*(1-TLC_revoke);
      |
      | Operative_Level=1-Mechanical_Fault;
      mask step_sended=|
      | TLC_CONN=Connection*Operative_Level;
      | TLC_SERVICE=TLC_services*Operative_Level+TLC_revoke*10;
      |
      |
      | CYBER_FAULT=Cyber_Fault*Operative_Level;
      | MECH_FAULT=Mechanical_Fault;
      mask prompts: Parameter1 "entity name"; Parameter2 "sampling time"; Parameter3 "project"; resources "input resources and state variables"; Parameter10 "Bring state variables to output"; codeupdate "update code from mask"
      mask help: This is a level-2 MATLAB file S-function which demonstrates CISIA entity
      mask DialogControl Container1 Prompt: All parameters
      mask Display: image('Icons/Optical_Wire.png')
  Wire_8 (21) : M-S-Function  FunctionName=cisia_msfun  Parameters=Parameter1, Parameter2, Parameter3, resources, Parameter10, codeupdate, step_received, step_computed, dynamic_computed, step_sended, id_entity, id_project, id_type, name_type, color  mask(S-function:msfcn_unit_delay){Parameter1='Wire_8', Parameter2=1, Parameter3='ORO', resources=|, Parameter10=off, codeupdate=off, step_received=|, step_computed=, dynamic_computed=, step_sended=|, id_entity=21, id_project=38, id_type=1, name_type=Optical_Wire, color=#99CCFF}
      mask resources=|
      | *** INPUT RESOURCES ***
      | NUM_INPUTS 4
      | TLC_CONN (20)
      | TLC_SERVICE (20)
      | CYBER_FAULT (10)
      | MECH_FAULT (1)
      |
      | *** STATE VARIABLES ***
      | NUM_VARIABLES 11
      | Operative_Level(NUMERIC)(1)(1)
      | TLC_services(NUMERIC_ARRAY)(20)(0  0  0  0  0  0  0  0  0  0  0  0  0  0  0  0  0  0  0  0)
      | Connection(NUMERIC_ARRAY)(20)(0  0  0  0  0  0  0  0  0  0  0  0  0  0  0  0  0  0  0  0)
      | Dos_attack(NUMERIC)(1)(0)
      | MITM_attack(NUMERIC)(1)(0)
      | Virus_Attack(NUMERIC)(1)(0)
      | Port_Scan_Attack(NUMERIC)(1)(0)
      | Cyber_Fault(NUMERIC_ARRAY)(10)(0  0  0  0  0  0  0  0  0  0)
      | Mechanical_Fault(NUMERIC)(1)(0)
      | Conn_Fault(NUMERIC)(1)(0)
      | TLC_revoke(NUMERIC_ARRAY)(20)(0  0  0  0  0  0  0  0  0  0  0  0  0  0  0  0  0  0  0  0)
      |
      | *** OUTPUT RESOURCES ***
      | NUM_OUTPUTS 4
      | TLC_CONN (20)
      | TLC_SERVICE (20)
      | CYBER_FAULT (10)
      | MECH_FAULT (1)
      mask step_received=|
      | Connection=max(Connection_init,TLC_CONN);
      | TLC_services=max(TLC_services_init,TLC_SERVICE);
      | TLC_services=mod(TLC_services,10);
      | TLC_revoke=floor(TLC_SERVICE/10);
      |
      | Cyber_Fault=CYBER_FAULT;
      |
      | Mechanical_Fault=max([Mechanical_Fault MECH_FAULT Mechanical_Fault_init]);
      |
      | %TLC_services=TLC_services.*(1-TLC_revoke);
      |
      | Operative_Level=1-Mechanical_Fault;
      mask step_sended=|
      | TLC_CONN=Connection*Operative_Level;
      | TLC_SERVICE=TLC_services*Operative_Level+TLC_revoke*10;
      |
      |
      | CYBER_FAULT=Cyber_Fault*Operative_Level;
      | MECH_FAULT=Mechanical_Fault;
      mask prompts: Parameter1 "entity name"; Parameter2 "sampling time"; Parameter3 "project"; resources "input resources and state variables"; Parameter10 "Bring state variables to output"; codeupdate "update code from mask"
      mask help: This is a level-2 MATLAB file S-function which demonstrates CISIA entity
      mask DialogControl Container1 Prompt: All parameters
      mask Display: image('Icons/Optical_Wire.png')
  Wire_8b (22) : M-S-Function  FunctionName=cisia_msfun  Parameters=Parameter1, Parameter2, Parameter3, resources, Parameter10, codeupdate, step_received, step_computed, dynamic_computed, step_sended, id_entity, id_project, id_type, name_type, color  mask(S-function:msfcn_unit_delay){Parameter1='Wire_8b', Parameter2=1, Parameter3='ORO', resources=|, Parameter10=off, codeupdate=off, step_received=|, step_computed=, dynamic_computed=, step_sended=|, id_entity=22, id_project=38, id_type=1, name_type=Optical_Wire, color=#99CCFF}
      mask resources=|
      | *** INPUT RESOURCES ***
      | NUM_INPUTS 4
      | TLC_CONN (20)
      | TLC_SERVICE (20)
      | CYBER_FAULT (10)
      | MECH_FAULT (1)
      |
      | *** STATE VARIABLES ***
      | NUM_VARIABLES 11
      | Operative_Level(NUMERIC)(1)(1)
      | TLC_services(NUMERIC_ARRAY)(20)(0  0  0  0  0  0  0  0  0  0  0  0  0  0  0  0  0  0  0  0)
      | Connection(NUMERIC_ARRAY)(20)(0  0  0  0  0  0  0  0  0  0  0  0  0  0  0  0  0  0  0  0)
      | Dos_attack(NUMERIC)(1)(0)
      | MITM_attack(NUMERIC)(1)(0)
      | Virus_Attack(NUMERIC)(1)(0)
      | Port_Scan_Attack(NUMERIC)(1)(0)
      | Cyber_Fault(NUMERIC_ARRAY)(10)(0  0  0  0  0  0  0  0  0  0)
      | Mechanical_Fault(NUMERIC)(1)(0)
      | Conn_Fault(NUMERIC)(1)(0)
      | TLC_revoke(NUMERIC_ARRAY)(20)(0  0  0  0  0  0  0  0  0  0  0  0  0  0  0  0  0  0  0  0)
      |
      | *** OUTPUT RESOURCES ***
      | NUM_OUTPUTS 4
      | TLC_CONN (20)
      | TLC_SERVICE (20)
      | CYBER_FAULT (10)
      | MECH_FAULT (1)
      mask step_received=|
      | Connection=max(Connection_init,TLC_CONN);
      | TLC_services=max(TLC_services_init,TLC_SERVICE);
      | TLC_services=mod(TLC_services,10);
      | TLC_revoke=floor(TLC_SERVICE/10);
      |
      | Cyber_Fault=CYBER_FAULT;
      |
      | Mechanical_Fault=max([Mechanical_Fault MECH_FAULT Mechanical_Fault_init]);
      |
      | %TLC_services=TLC_services.*(1-TLC_revoke);
      |
      | Operative_Level=1-Mechanical_Fault;
      mask step_sended=|
      | TLC_CONN=Connection*Operative_Level;
      | TLC_SERVICE=TLC_services*Operative_Level+TLC_revoke*10;
      |
      |
      | CYBER_FAULT=Cyber_Fault*Operative_Level;
      | MECH_FAULT=Mechanical_Fault;
      mask prompts: Parameter1 "entity name"; Parameter2 "sampling time"; Parameter3 "project"; resources "input resources and state variables"; Parameter10 "Bring state variables to output"; codeupdate "update code from mask"
      mask help: This is a level-2 MATLAB file S-function which demonstrates CISIA entity
      mask DialogControl Container1 Prompt: All parameters
      mask Display: image('Icons/Optical_Wire.png')
  Wire_9 (28) : M-S-Function  FunctionName=cisia_msfun  Parameters=Parameter1, Parameter2, Parameter3, resources, Parameter10, codeupdate, step_received, step_computed, dynamic_computed, step_sended, id_entity, id_project, id_type, name_type, color  mask(S-function:msfcn_unit_delay){Parameter1='Wire_9', Parameter2=1, Parameter3='ORO', resources=|, Parameter10=off, codeupdate=off, step_received=|, step_computed=, dynamic_computed=, step_sended=|, id_entity=28, id_project=38, id_type=1, name_type=Optical_Wire, color=#99CCFF}
      mask resources=|
      | *** INPUT RESOURCES ***
      | NUM_INPUTS 4
      | TLC_CONN (20)
      | TLC_SERVICE (20)
      | CYBER_FAULT (10)
      | MECH_FAULT (1)
      |
      | *** STATE VARIABLES ***
      | NUM_VARIABLES 11
      | Operative_Level(NUMERIC)(1)(1)
      | TLC_services(NUMERIC_ARRAY)(20)(0  0  0  0  0  0  0  0  0  0  0  0  0  0  0  0  0  0  0  0)
      | Connection(NUMERIC_ARRAY)(20)(0  0  0  0  0  0  0  0  0  0  0  0  0  0  0  0  0  0  0  0)
      | Dos_attack(NUMERIC)(1)(0)
      | MITM_attack(NUMERIC)(1)(0)
      | Virus_Attack(NUMERIC)(1)(0)
      | Port_Scan_Attack(NUMERIC)(1)(0)
      | Cyber_Fault(NUMERIC_ARRAY)(10)(0  0  0  0  0  0  0  0  0  0)
      | Mechanical_Fault(NUMERIC)(1)(0)
      | Conn_Fault(NUMERIC)(1)(0)
      | TLC_revoke(NUMERIC_ARRAY)(20)(0  0  0  0  0  0  0  0  0  0  0  0  0  0  0  0  0  0  0  0)
      |
      | *** OUTPUT RESOURCES ***
      | NUM_OUTPUTS 4
      | TLC_CONN (20)
      | TLC_SERVICE (20)
      | CYBER_FAULT (10)
      | MECH_FAULT (1)
      mask step_received=|
      | Connection=max(Connection_init,TLC_CONN);
      | TLC_services=max(TLC_services_init,TLC_SERVICE);
      | TLC_services=mod(TLC_services,10);
      | TLC_revoke=floor(TLC_SERVICE/10);
      |
      | Cyber_Fault=CYBER_FAULT;
      |
      | Mechanical_Fault=max([Mechanical_Fault MECH_FAULT Mechanical_Fault_init]);
      |
      | %TLC_services=TLC_services.*(1-TLC_revoke);
      |
      | Operative_Level=1-Mechanical_Fault;
      mask step_sended=|
      | TLC_CONN=Connection*Operative_Level;
      | TLC_SERVICE=TLC_services*Operative_Level+TLC_revoke*10;
      |
      |
      | CYBER_FAULT=Cyber_Fault*Operative_Level;
      | MECH_FAULT=Mechanical_Fault;
      mask prompts: Parameter1 "entity name"; Parameter2 "sampling time"; Parameter3 "project"; resources "input resources and state variables"; Parameter10 "Bring state variables to output"; codeupdate "update code from mask"
      mask help: This is a level-2 MATLAB file S-function which demonstrates CISIA entity
      mask DialogControl Container1 Prompt: All parameters
      mask Display: image('Icons/Optical_Wire.png')
  Wire_9b (29) : M-S-Function  FunctionName=cisia_msfun  Parameters=Parameter1, Parameter2, Parameter3, resources, Parameter10, codeupdate, step_received, step_computed, dynamic_computed, step_sended, id_entity, id_project, id_type, name_type, color  mask(S-function:msfcn_unit_delay){Parameter1='Wire_9b', Parameter2=1, Parameter3='ORO', resources=|, Parameter10=off, codeupdate=off, step_received=|, step_computed=, dynamic_computed=, step_sended=|, id_entity=29, id_project=38, id_type=1, name_type=Optical_Wire, color=#99CCFF}
      mask resources=|
      | *** INPUT RESOURCES ***
      | NUM_INPUTS 4
      | TLC_CONN (20)
      | TLC_SERVICE (20)
      | CYBER_FAULT (10)
      | MECH_FAULT (1)
      |
      | *** STATE VARIABLES ***
      | NUM_VARIABLES 11
      | Operative_Level(NUMERIC)(1)(1)
      | TLC_services(NUMERIC_ARRAY)(20)(0  0  0  0  0  0  0  0  0  0  0  0  0  0  0  0  0  0  0  0)
      | Connection(NUMERIC_ARRAY)(20)(0  0  0  0  0  0  0  0  0  0  0  0  0  0  0  0  0  0  0  0)
      | Dos_attack(NUMERIC)(1)(0)
      | MITM_attack(NUMERIC)(1)(0)
      | Virus_Attack(NUMERIC)(1)(0)
      | Port_Scan_Attack(NUMERIC)(1)(0)
      | Cyber_Fault(NUMERIC_ARRAY)(10)(0  0  0  0  0  0  0  0  0  0)
      | Mechanical_Fault(NUMERIC)(1)(0)
      | Conn_Fault(NUMERIC)(1)(0)
      | TLC_revoke(NUMERIC_ARRAY)(20)(0  0  0  0  0  0  0  0  0  0  0  0  0  0  0  0  0  0  0  0)
      |
      | *** OUTPUT RESOURCES ***
      | NUM_OUTPUTS 4
      | TLC_CONN (20)
      | TLC_SERVICE (20)
      | CYBER_FAULT (10)
      | MECH_FAULT (1)
      mask step_received=|
      | Connection=max(Connection_init,TLC_CONN);
      | TLC_services=max(TLC_services_init,TLC_SERVICE);
      | TLC_services=mod(TLC_services,10);
      | TLC_revoke=floor(TLC_SERVICE/10);
      |
      | Cyber_Fault=CYBER_FAULT;
      |
      | Mechanical_Fault=max([Mechanical_Fault MECH_FAULT Mechanical_Fault_init]);
      |
      | %TLC_services=TLC_services.*(1-TLC_revoke);
      |
      | Operative_Level=1-Mechanical_Fault;
      mask step_sended=|
      | TLC_CONN=Connection*Operative_Level;
      | TLC_SERVICE=TLC_services*Operative_Level+TLC_revoke*10;
      |
      |
      | CYBER_FAULT=Cyber_Fault*Operative_Level;
      | MECH_FAULT=Mechanical_Fault;
      mask prompts: Parameter1 "entity name"; Parameter2 "sampling time"; Parameter3 "project"; resources "input resources and state variables"; Parameter10 "Bring state variables to output"; codeupdate "update code from mask"
      mask help: This is a level-2 MATLAB file S-function which demonstrates CISIA entity
      mask DialogControl Container1 Prompt: All parameters
      mask Display: image('Icons/Optical_Wire.png')
  Wire_MR_1 (118) : M-S-Function  FunctionName=cisia_msfun  Parameters=Parameter1, Parameter2, Parameter3, resources, Parameter10, codeupdate, step_received, step_computed, dynamic_computed, step_sended, id_entity, id_project, id_type, name_type, color  mask(S-function:msfcn_unit_delay){Parameter1='Wire_MR_1', Parameter2=1, Parameter3='ORO', resources=|, Parameter10=off, codeupdate=off, step_received=|, step_computed=, dynamic_computed=, step_sended=|, id_entity=118, id_project=38, id_type=29, name_type=Wire_Medical_Room, color=#FFDD00}
      mask resources=|
      | *** INPUT RESOURCES ***
      | NUM_INPUTS 1
      | POWER (1)
      |
      | *** STATE VARIABLES ***
      | NUM_VARIABLES 3
      | Operative_Level(NUMERIC)(1)(1)
      | Mechanical_Fault(NUMERIC)(1)(0)
      | Power_Fault(NUMERIC)(1)(0)
      |
      | *** OUTPUT RESOURCES ***
      | NUM_OUTPUTS 2
      | POWER (1)
      | WIRE_QoS (1)
      mask step_received=|
      | Power_Fault=1-POWER;
      |
      | Operative_Level = (1-Mechanical_Fault)*(1-0.5*Power_Fault);
      mask step_sended=|
      | POWER=Operative_Level;
      | WIRE_QoS=Operative_Level;
      mask prompts: Parameter1 "entity name"; Parameter2 "sampling time"; Parameter3 "project"; resources "input resources and state variables"; Parameter10 "Bring state variables to output"; codeupdate "update code from mask"
      mask help: This is a level-2 MATLAB file S-function which demonstrates CISIA entity
      mask DialogControl Container1 Prompt: All parameters
      mask Display: disp('Wire_Medical_Room')
  Wire_MR_2 (136) : M-S-Function  FunctionName=cisia_msfun  Parameters=Parameter1, Parameter2, Parameter3, resources, Parameter10, codeupdate, step_received, step_computed, dynamic_computed, step_sended, id_entity, id_project, id_type, name_type, color  mask(S-function:msfcn_unit_delay){Parameter1='Wire_MR_2', Parameter2=1, Parameter3='ORO', resources=|, Parameter10=off, codeupdate=off, step_received=|, step_computed=, dynamic_computed=, step_sended=|, id_entity=136, id_project=38, id_type=29, name_type=Wire_Medical_Room, color=#FFDD00}
      mask resources=|
      | *** INPUT RESOURCES ***
      | NUM_INPUTS 1
      | POWER (1)
      |
      | *** STATE VARIABLES ***
      | NUM_VARIABLES 3
      | Operative_Level(NUMERIC)(1)(1)
      | Mechanical_Fault(NUMERIC)(1)(0)
      | Power_Fault(NUMERIC)(1)(0)
      |
      | *** OUTPUT RESOURCES ***
      | NUM_OUTPUTS 2
      | POWER (1)
      | WIRE_QoS (1)
      mask step_received=|
      | Power_Fault=1-POWER;
      |
      | Operative_Level = (1-Mechanical_Fault)*(1-0.5*Power_Fault);
      mask step_sended=|
      | POWER=Operative_Level;
      | WIRE_QoS=Operative_Level;
      mask prompts: Parameter1 "entity name"; Parameter2 "sampling time"; Parameter3 "project"; resources "input resources and state variables"; Parameter10 "Bring state variables to output"; codeupdate "update code from mask"
      mask help: This is a level-2 MATLAB file S-function which demonstrates CISIA entity
      mask DialogControl Container1 Prompt: All parameters
      mask Display: disp('Wire_Medical_Room')
  Wire_MR_3 (137) : M-S-Function  FunctionName=cisia_msfun  Parameters=Parameter1, Parameter2, Parameter3, resources, Parameter10, codeupdate, step_received, step_computed, dynamic_computed, step_sended, id_entity, id_project, id_type, name_type, color  mask(S-function:msfcn_unit_delay){Parameter1='Wire_MR_3', Parameter2=1, Parameter3='ORO', resources=|, Parameter10=off, codeupdate=off, step_received=|, step_computed=, dynamic_computed=, step_sended=|, id_entity=137, id_project=38, id_type=29, name_type=Wire_Medical_Room, color=#FFDD00}
      mask resources=|
      | *** INPUT RESOURCES ***
      | NUM_INPUTS 1
      | POWER (1)
      |
      | *** STATE VARIABLES ***
      | NUM_VARIABLES 3
      | Operative_Level(NUMERIC)(1)(1)
      | Mechanical_Fault(NUMERIC)(1)(0)
      | Power_Fault(NUMERIC)(1)(0)
      |
      | *** OUTPUT RESOURCES ***
      | NUM_OUTPUTS 2
      | POWER (1)
      | WIRE_QoS (1)
      mask step_received=|
      | Power_Fault=1-POWER;
      |
      | Operative_Level = (1-Mechanical_Fault)*(1-0.5*Power_Fault);
      mask step_sended=|
      | POWER=Operative_Level;
      | WIRE_QoS=Operative_Level;
      mask prompts: Parameter1 "entity name"; Parameter2 "sampling time"; Parameter3 "project"; resources "input resources and state variables"; Parameter10 "Bring state variables to output"; codeupdate "update code from mask"
      mask help: This is a level-2 MATLAB file S-function which demonstrates CISIA entity
      mask DialogControl Container1 Prompt: All parameters
      mask Display: disp('Wire_Medical_Room')
  Wire_MR_4 (138) : M-S-Function  FunctionName=cisia_msfun  Parameters=Parameter1, Parameter2, Parameter3, resources, Parameter10, codeupdate, step_received, step_computed, dynamic_computed, step_sended, id_entity, id_project, id_type, name_type, color  mask(S-function:msfcn_unit_delay){Parameter1='Wire_MR_4', Parameter2=1, Parameter3='ORO', resources=|, Parameter10=off, codeupdate=off, step_received=|, step_computed=, dynamic_computed=, step_sended=|, id_entity=138, id_project=38, id_type=29, name_type=Wire_Medical_Room, color=#FFDD00}
      mask resources=|
      | *** INPUT RESOURCES ***
      | NUM_INPUTS 1
      | POWER (1)
      |
      | *** STATE VARIABLES ***
      | NUM_VARIABLES 3
      | Operative_Level(NUMERIC)(1)(1)
      | Mechanical_Fault(NUMERIC)(1)(0)
      | Power_Fault(NUMERIC)(1)(0)
      |
      | *** OUTPUT RESOURCES ***
      | NUM_OUTPUTS 2
      | POWER (1)
      | WIRE_QoS (1)
      mask step_received=|
      | Power_Fault=1-POWER;
      |
      | Operative_Level = (1-Mechanical_Fault)*(1-0.5*Power_Fault);
      mask step_sended=|
      | POWER=Operative_Level;
      | WIRE_QoS=Operative_Level;
      mask prompts: Parameter1 "entity name"; Parameter2 "sampling time"; Parameter3 "project"; resources "input resources and state variables"; Parameter10 "Bring state variables to output"; codeupdate "update code from mask"
      mask help: This is a level-2 MATLAB file S-function which demonstrates CISIA entity
      mask DialogControl Container1 Prompt: All parameters
      mask Display: disp('Wire_Medical_Room')
  Wire_MR_5 (139) : M-S-Function  FunctionName=cisia_msfun  Parameters=Parameter1, Parameter2, Parameter3, resources, Parameter10, codeupdate, step_received, step_computed, dynamic_computed, step_sended, id_entity, id_project, id_type, name_type, color  mask(S-function:msfcn_unit_delay){Parameter1='Wire_MR_5', Parameter2=1, Parameter3='ORO', resources=|, Parameter10=off, codeupdate=off, step_received=|, step_computed=, dynamic_computed=, step_sended=|, id_entity=139, id_project=38, id_type=29, name_type=Wire_Medical_Room, color=#FFDD00}
      mask resources=|
      | *** INPUT RESOURCES ***
      | NUM_INPUTS 1
      | POWER (1)
      |
      | *** STATE VARIABLES ***
      | NUM_VARIABLES 3
      | Operative_Level(NUMERIC)(1)(1)
      | Mechanical_Fault(NUMERIC)(1)(0)
      | Power_Fault(NUMERIC)(1)(0)
      |
      | *** OUTPUT RESOURCES ***
      | NUM_OUTPUTS 2
      | POWER (1)
      | WIRE_QoS (1)
      mask step_received=|
      | Power_Fault=1-POWER;
      |
      | Operative_Level = (1-Mechanical_Fault)*(1-0.5*Power_Fault);
      mask step_sended=|
      | POWER=Operative_Level;
      | WIRE_QoS=Operative_Level;
      mask prompts: Parameter1 "entity name"; Parameter2 "sampling time"; Parameter3 "project"; resources "input resources and state variables"; Parameter10 "Bring state variables to output"; codeupdate "update code from mask"
      mask help: This is a level-2 MATLAB file S-function which demonstrates CISIA entity
      mask DialogControl Container1 Prompt: All parameters
      mask Display: disp('Wire_Medical_Room')
  Wire_MR_6 (140) : M-S-Function  FunctionName=cisia_msfun  Parameters=Parameter1, Parameter2, Parameter3, resources, Parameter10, codeupdate, step_received, step_computed, dynamic_computed, step_sended, id_entity, id_project, id_type, name_type, color  mask(S-function:msfcn_unit_delay){Parameter1='Wire_MR_6', Parameter2=1, Parameter3='ORO', resources=|, Parameter10=off, codeupdate=off, step_received=|, step_computed=, dynamic_computed=, step_sended=|, id_entity=140, id_project=38, id_type=29, name_type=Wire_Medical_Room, color=#FFDD00}
      mask resources=|
      | *** INPUT RESOURCES ***
      | NUM_INPUTS 1
      | POWER (1)
      |
      | *** STATE VARIABLES ***
      | NUM_VARIABLES 3
      | Operative_Level(NUMERIC)(1)(1)
      | Mechanical_Fault(NUMERIC)(1)(0)
      | Power_Fault(NUMERIC)(1)(0)
      |
      | *** OUTPUT RESOURCES ***
      | NUM_OUTPUTS 2
      | POWER (1)
      | WIRE_QoS (1)
      mask step_received=|
      | Power_Fault=1-POWER;
      |
      | Operative_Level = (1-Mechanical_Fault)*(1-0.5*Power_Fault);
      mask step_sended=|
      | POWER=Operative_Level;
      | WIRE_QoS=Operative_Level;
      mask prompts: Parameter1 "entity name"; Parameter2 "sampling time"; Parameter3 "project"; resources "input resources and state variables"; Parameter10 "Bring state variables to output"; codeupdate "update code from mask"
      mask help: This is a level-2 MATLAB file S-function which demonstrates CISIA entity
      mask DialogControl Container1 Prompt: All parameters
      mask Display: disp('Wire_Medical_Room')
  Wire_OP_1 (161) : M-S-Function  FunctionName=cisia_msfun  Parameters=Parameter1, Parameter2, Parameter3, resources, Parameter10, codeupdate, step_received, step_computed, dynamic_computed, step_sended, id_entity, id_project, id_type, name_type, color  mask(S-function:msfcn_unit_delay){Parameter1='Wire_OP_1', Parameter2=1, Parameter3='ORO', resources=|, Parameter10=off, codeupdate=off, step_received=|, step_computed=, dynamic_computed=, step_sended=|, id_entity=161, id_project=38, id_type=29, name_type=Wire_Medical_Room, color=#FFDD00}
      mask resources=|
      | *** INPUT RESOURCES ***
      | NUM_INPUTS 1
      | POWER (1)
      |
      | *** STATE VARIABLES ***
      | NUM_VARIABLES 3
      | Operative_Level(NUMERIC)(1)(1)
      | Mechanical_Fault(NUMERIC)(1)(0)
      | Power_Fault(NUMERIC)(1)(0)
      |
      | *** OUTPUT RESOURCES ***
      | NUM_OUTPUTS 2
      | POWER (1)
      | WIRE_QoS (1)
      mask step_received=|
      | Power_Fault=1-POWER;
      |
      | Operative_Level = (1-Mechanical_Fault)*(1-0.5*Power_Fault);
      mask step_sended=|
      | POWER=Operative_Level;
      | WIRE_QoS=Operative_Level;
      mask prompts: Parameter1 "entity name"; Parameter2 "sampling time"; Parameter3 "project"; resources "input resources and state variables"; Parameter10 "Bring state variables to output"; codeupdate "update code from mask"
      mask help: This is a level-2 MATLAB file S-function which demonstrates CISIA entity
      mask DialogControl Container1 Prompt: All parameters
      mask Display: disp('Wire_Medical_Room')
  Wire_OP_2 (162) : M-S-Function  FunctionName=cisia_msfun  Parameters=Parameter1, Parameter2, Parameter3, resources, Parameter10, codeupdate, step_received, step_computed, dynamic_computed, step_sended, id_entity, id_project, id_type, name_type, color  mask(S-function:msfcn_unit_delay){Parameter1='Wire_OP_2', Parameter2=1, Parameter3='ORO', resources=|, Parameter10=off, codeupdate=off, step_received=|, step_computed=, dynamic_computed=, step_sended=|, id_entity=162, id_project=38, id_type=29, name_type=Wire_Medical_Room, color=#FFDD00}
      mask resources=|
      | *** INPUT RESOURCES ***
      | NUM_INPUTS 1
      | POWER (1)
      |
      | *** STATE VARIABLES ***
      | NUM_VARIABLES 3
      | Operative_Level(NUMERIC)(1)(1)
      | Mechanical_Fault(NUMERIC)(1)(0)
      | Power_Fault(NUMERIC)(1)(0)
      |
      | *** OUTPUT RESOURCES ***
      | NUM_OUTPUTS 2
      | POWER (1)
      | WIRE_QoS (1)
      mask step_received=|
      | Power_Fault=1-POWER;
      |
      | Operative_Level = (1-Mechanical_Fault)*(1-0.5*Power_Fault);
      mask step_sended=|
      | POWER=Operative_Level;
      | WIRE_QoS=Operative_Level;
      mask prompts: Parameter1 "entity name"; Parameter2 "sampling time"; Parameter3 "project"; resources "input resources and state variables"; Parameter10 "Bring state variables to output"; codeupdate "update code from mask"
      mask help: This is a level-2 MATLAB file S-function which demonstrates CISIA entity
      mask DialogControl Container1 Prompt: All parameters
      mask Display: disp('Wire_Medical_Room')
  Wire_OR_1 (163) : M-S-Function  FunctionName=cisia_msfun  Parameters=Parameter1, Parameter2, Parameter3, resources, Parameter10, codeupdate, step_received, step_computed, dynamic_computed, step_sended, id_entity, id_project, id_type, name_type, color  mask(S-function:msfcn_unit_delay){Parameter1='Wire_OR_1', Parameter2=1, Parameter3='ORO', resources=|, Parameter10=off, codeupdate=off, step_received=|, step_computed=, dynamic_computed=, step_sended=|, id_entity=163, id_project=38, id_type=29, name_type=Wire_Medical_Room, color=#FFDD00}
      mask resources=|
      | *** INPUT RESOURCES ***
      | NUM_INPUTS 1
      | POWER (1)
      |
      | *** STATE VARIABLES ***
      | NUM_VARIABLES 3
      | Operative_Level(NUMERIC)(1)(1)
      | Mechanical_Fault(NUMERIC)(1)(0)
      | Power_Fault(NUMERIC)(1)(0)
      |
      | *** OUTPUT RESOURCES ***
      | NUM_OUTPUTS 2
      | POWER (1)
      | WIRE_QoS (1)
      mask step_received=|
      | Power_Fault=1-POWER;
      |
      | Operative_Level = (1-Mechanical_Fault)*(1-0.5*Power_Fault);
      mask step_sended=|
      | POWER=Operative_Level;
      | WIRE_QoS=Operative_Level;
      mask prompts: Parameter1 "entity name"; Parameter2 "sampling time"; Parameter3 "project"; resources "input resources and state variables"; Parameter10 "Bring state variables to output"; codeupdate "update code from mask"
      mask help: This is a level-2 MATLAB file S-function which demonstrates CISIA entity
      mask DialogControl Container1 Prompt: All parameters
      mask Display: disp('Wire_Medical_Room')
  Wire_OR_2 (164) : M-S-Function  FunctionName=cisia_msfun  Parameters=Parameter1, Parameter2, Parameter3, resources, Parameter10, codeupdate, step_received, step_computed, dynamic_computed, step_sended, id_entity, id_project, id_type, name_type, color  mask(S-function:msfcn_unit_delay){Parameter1='Wire_OR_2', Parameter2=1, Parameter3='ORO', resources=|, Parameter10=off, codeupdate=off, step_received=|, step_computed=, dynamic_computed=, step_sended=|, id_entity=164, id_project=38, id_type=29, name_type=Wire_Medical_Room, color=#FFDD00}
      mask resources=|
      | *** INPUT RESOURCES ***
      | NUM_INPUTS 1
      | POWER (1)
      |
      | *** STATE VARIABLES ***
      | NUM_VARIABLES 3
      | Operative_Level(NUMERIC)(1)(1)
      | Mechanical_Fault(NUMERIC)(1)(0)
      | Power_Fault(NUMERIC)(1)(0)
      |
      | *** OUTPUT RESOURCES ***
      | NUM_OUTPUTS 2
      | POWER (1)
      | WIRE_QoS (1)
      mask step_received=|
      | Power_Fault=1-POWER;
      |
      | Operative_Level = (1-Mechanical_Fault)*(1-0.5*Power_Fault);
      mask step_sended=|
      | POWER=Operative_Level;
      | WIRE_QoS=Operative_Level;
      mask prompts: Parameter1 "entity name"; Parameter2 "sampling time"; Parameter3 "project"; resources "input resources and state variables"; Parameter10 "Bring state variables to output"; codeupdate "update code from mask"
      mask help: This is a level-2 MATLAB file S-function which demonstrates CISIA entity
      mask DialogControl Container1 Prompt: All parameters
      mask Display: disp('Wire_Medical_Room')
  Wire_OR_3 (165) : M-S-Function  FunctionName=cisia_msfun  Parameters=Parameter1, Parameter2, Parameter3, resources, Parameter10, codeupdate, step_received, step_computed, dynamic_computed, step_sended, id_entity, id_project, id_type, name_type, color  mask(S-function:msfcn_unit_delay){Parameter1='Wire_OR_3', Parameter2=1, Parameter3='ORO', resources=|, Parameter10=off, codeupdate=off, step_received=|, step_computed=, dynamic_computed=, step_sended=|, id_entity=165, id_project=38, id_type=29, name_type=Wire_Medical_Room, color=#FFDD00}
      mask resources=|
      | *** INPUT RESOURCES ***
      | NUM_INPUTS 1
      | POWER (1)
      |
      | *** STATE VARIABLES ***
      | NUM_VARIABLES 3
      | Operative_Level(NUMERIC)(1)(1)
      | Mechanical_Fault(NUMERIC)(1)(0)
      | Power_Fault(NUMERIC)(1)(0)
      |
      | *** OUTPUT RESOURCES ***
      | NUM_OUTPUTS 2
      | POWER (1)
      | WIRE_QoS (1)
      mask step_received=|
      | Power_Fault=1-POWER;
      |
      | Operative_Level = (1-Mechanical_Fault)*(1-0.5*Power_Fault);
      mask step_sended=|
      | POWER=Operative_Level;
      | WIRE_QoS=Operative_Level;
      mask prompts: Parameter1 "entity name"; Parameter2 "sampling time"; Parameter3 "project"; resources "input resources and state variables"; Parameter10 "Bring state variables to output"; codeupdate "update code from mask"
      mask help: This is a level-2 MATLAB file S-function which demonstrates CISIA entity
      mask DialogControl Container1 Prompt: All parameters
      mask Display: disp('Wire_Medical_Room')
  Wire_S_1 (166) : M-S-Function  FunctionName=cisia_msfun  Parameters=Parameter1, Parameter2, Parameter3, resources, Parameter10, codeupdate, step_received, step_computed, dynamic_computed, step_sended, id_entity, id_project, id_type, name_type, color  mask(S-function:msfcn_unit_delay){Parameter1='Wire_S_1', Parameter2=1, Parameter3='ORO', resources=|, Parameter10=off, codeupdate=off, step_received=|, step_computed=, dynamic_computed=, step_sended=|, id_entity=166, id_project=38, id_type=29, name_type=Wire_Medical_Room, color=#FFDD00}
      mask resources=|
      | *** INPUT RESOURCES ***
      | NUM_INPUTS 1
      | POWER (1)
      |
      | *** STATE VARIABLES ***
      | NUM_VARIABLES 3
      | Operative_Level(NUMERIC)(1)(1)
      | Mechanical_Fault(NUMERIC)(1)(0)
      | Power_Fault(NUMERIC)(1)(0)
      |
      | *** OUTPUT RESOURCES ***
      | NUM_OUTPUTS 2
      | POWER (1)
      | WIRE_QoS (1)
      mask step_received=|
      | Power_Fault=1-POWER;
      |
      | Operative_Level = (1-Mechanical_Fault)*(1-0.5*Power_Fault);
      mask step_sended=|
      | POWER=Operative_Level;
      | WIRE_QoS=Operative_Level;
      mask prompts: Parameter1 "entity name"; Parameter2 "sampling time"; Parameter3 "project"; resources "input resources and state variables"; Parameter10 "Bring state variables to output"; codeupdate "update code from mask"
      mask help: This is a level-2 MATLAB file S-function which demonstrates CISIA entity
      mask DialogControl Container1 Prompt: All parameters
      mask Display: disp('Wire_Medical_Room')
  Wire_S_2 (167) : M-S-Function  FunctionName=cisia_msfun  Parameters=Parameter1, Parameter2, Parameter3, resources, Parameter10, codeupdate, step_received, step_computed, dynamic_computed, step_sended, id_entity, id_project, id_type, name_type, color  mask(S-function:msfcn_unit_delay){Parameter1='Wire_S_2', Parameter2=1, Parameter3='ORO', resources=|, Parameter10=off, codeupdate=off, step_received=|, step_computed=, dynamic_computed=, step_sended=|, id_entity=167, id_project=38, id_type=29, name_type=Wire_Medical_Room, color=#FFDD00}
      mask resources=|
      | *** INPUT RESOURCES ***
      | NUM_INPUTS 1
      | POWER (1)
      |
      | *** STATE VARIABLES ***
      | NUM_VARIABLES 3
      | Operative_Level(NUMERIC)(1)(1)
      | Mechanical_Fault(NUMERIC)(1)(0)
      | Power_Fault(NUMERIC)(1)(0)
      |
      | *** OUTPUT RESOURCES ***
      | NUM_OUTPUTS 2
      | POWER (1)
      | WIRE_QoS (1)
      mask step_received=|
      | Power_Fault=1-POWER;
      |
      | Operative_Level = (1-Mechanical_Fault)*(1-0.5*Power_Fault);
      mask step_sended=|
      | POWER=Operative_Level;
      | WIRE_QoS=Operative_Level;
      mask prompts: Parameter1 "entity name"; Parameter2 "sampling time"; Parameter3 "project"; resources "input resources and state variables"; Parameter10 "Bring state variables to output"; codeupdate "update code from mask"
      mask help: This is a level-2 MATLAB file S-function which demonstrates CISIA entity
      mask DialogControl Container1 Prompt: All parameters
      mask Display: disp('Wire_Medical_Room')
  media : MATLAB Function  TreatAsAtomicUnit=on
  media1 : MATLAB Function  TreatAsAtomicUnit=on
  media10 : MATLAB Function  TreatAsAtomicUnit=on
  media11 : MATLAB Function  TreatAsAtomicUnit=on
  media12 : MATLAB Function  TreatAsAtomicUnit=on
  media13 : MATLAB Function  TreatAsAtomicUnit=on
  media2 : MATLAB Function  TreatAsAtomicUnit=on
  media3 : MATLAB Function  TreatAsAtomicUnit=on
  media4 : MATLAB Function  TreatAsAtomicUnit=on
  media5 : MATLAB Function  TreatAsAtomicUnit=on
  media6 : MATLAB Function  TreatAsAtomicUnit=on
  media7 : MATLAB Function  TreatAsAtomicUnit=on
  media8 : MATLAB Function  TreatAsAtomicUnit=on
  media9 : MATLAB Function  TreatAsAtomicUnit=on
  wires:
  Wire_8 (21)/4 -> Wire_8b (22)/4  "MECH_FAULT"
  ASR920_1 (7)/4 -> [Routing_QoS_920_1]  "ROUTING_QoS"
  ASR9006_2 (10)/2 -> Wire_7 (19)/2, Wire_2b (97)/2, Wire_3 (11)/2  "TLC_SERVICE"
  Wire_14 (42)/4 -> Wire_14b (43)/4  "MECH_FAULT"
  Wire_9 (28)/4 -> Wire_9b (29)/4  "MECH_FAULT"
  Wire_7b (20)/4 -> Wire_7 (19)/4  "MECH_FAULT"
  ASR920_1 (7)/2 -> Wire_6b (18)/2, Wire_14 (42)/2, Wire_12 (38)/2, Wire_15 (44)/2  "TLC_SERVICE"
  Wire_8b (22)/4 -> Wire_8 (21)/4  "MECH_FAULT"
  Wire_12 (38)/4 -> Wire_12b (39)/4  "MECH_FAULT"
  Wire_10 (30)/4 -> Wire_10b (31)/4  "MECH_FAULT"
  ASR9006_1 (9)/4 -> [Routing_QoS_9006_1]  "ROUTING_QoS"
  Wire_4 (12)/4 -> Wire_4b (13)/4  "MECH_FAULT"
  ASR903_2 (6)/4 -> [Routing_QoS_903_2]  "ROUTING_QoS"
  [POWER_1] -> ASR9006_1 (9)/4  "POWER"
  Wire_7 (19)/4 -> Wire_7b (20)/4  "MECH_FAULT"
  ASR903_2 (6)/1 -> Wire_5 (15)/1, Wire_9 (28)/1, Wire_3b (14)/1  "TLC_CONN"
  FG1500_1 (32)/4 -> [FW_QoS_1]  "FIREWALL_QoS"
  Nex_1 (3)/2 -> ROUTE_TIM_1 (20)/1  "TLC_SERVICE"
  [Room_QoS_2] -> Nex_2 (4)/5  "ROOM_QoS"
  [Room_QoS_2] -> ASR9006_2 (10)/5  "ROOM_QoS"
  [Room_QoS_1] -> Nex_1 (3)/5  "ROOM_QoS"
  Room_11 (258)/1 -> FG1500_1 (32)/5, BIGP_1 (34)/5  "ROOM_QoS"
  Nex_1 (3)/1 -> Wire_8 (21)/1, Wire_2 (2)/1, R_Wire_1 (98)/1  "TLC_CONN"
  Wire_12b (39)/4 -> Wire_12 (38)/4  "MECH_FAULT"
  BIGP_1 (34)/3 -> Wire_14b (43)/3  "CYBER_FAULT"
  Wire_3 (11)/4 -> Wire_3b (14)/4  "MECH_FAULT"
  Nex_2 (4)/2 -> ROUTE_TIM_2 (21)/1  "TLC_SERVICE"
  Wire_6 (17)/4 -> Wire_6b (18)/4  "MECH_FAULT"
  [POWER_2] -> ASR9006_2 (10)/4  "POWER"
  FG1500_1 (32)/5 -> [Redundancy_QoS_FG1500_2]  "REDUNDANCY_QoS"
  Wire_9b (29)/4 -> Wire_9 (28)/4  "MECH_FAULT"
  ASR920_2 (8)/1 -> Wire_18 (190)/1, Wire_17b (188)/1, Wire_11b (37)/1, Wire_5b (16)/1  "TLC_CONN"
  BIGP_1 (34)/1 -> Wire_14b (43)/1  "TLC_CONN"
  TLC_service2/1 -> Nex_1 (3)/2  "TLC_SERVICE"
  TLC_service1/1 -> Nex_2 (4)/2  "TLC_SERVICE"
  TLC_conn2/1 -> Nex_1 (3)/1  "TLC_CONN"
  Wire_14b (43)/4 -> Wire_14 (42)/4  "MECH_FAULT"
  Wire_5 (15)/4 -> Wire_5b (16)/4  "MECH_FAULT"
  Alcatel_1 (26)/1 -> Wire_10 (30)/1, 5G_Core_1 (198)/1, Cloud_Roma (238)/1  "TLC_CONN"
  ASR9006_1 (9)/2 -> Wire_4b (13)/2, Wire_1b (96)/2, Wire_8b (22)/2  "TLC_SERVICE"
  ASR9006_2 (10)/1 -> Wire_3 (11)/1, Wire_7 (19)/1, Wire_2b (97)/1  "TLC_CONN"
  ASR9006_1 (9)/1 -> Wire_4b (13)/1, Wire_1b (96)/1, Wire_8b (22)/1  "TLC_CONN"
  ASR903_2 (6)/3 -> Wire_5 (15)/3, Wire_9 (28)/3, Wire_3b (14)/3  "CYBER_FAULT"
  ASR920_1 (7)/1 -> Wire_6b (18)/1, Wire_14 (42)/1, Wire_12 (38)/1, Wire_15 (44)/1  "TLC_CONN"
  CYBER_fault2/1 -> Nex_1 (3)/3  "CYBER_FAULT"
  R_Wire_1 (98)/2 -> TLC_service1/1  "TLC_SERVICE"
  [Room_QoS_1] -> ASR9006_1 (9)/5  "ROOM_QoS"
  ASR903_1 (5)/2 -> Wire_10b (31)/2, Wire_4 (12)/2, Wire_6 (17)/2  "TLC_SERVICE"
  ASR9006_2 (10)/4 -> [Routing_QoS_9006_2]  "ROUTING_QoS"
  [POWER_1] -> Nex_1 (3)/4  "POWER"
  [POWER_2] -> Nex_2 (4)/4  "POWER"
  [POWER_4] -> Room_11 (258)/1, FG1500_1 (32)/4, BIGP_1 (34)/4  "POWER"
  TLC_conn1/1 -> Nex_2 (4)/1  "TLC_CONN"
  ASR903_1 (5)/4 -> [Routing_QoS_903_1]  "ROUTING_QoS"
  ASR903_1 (5)/3 -> Wire_4 (12)/3, Wire_6 (17)/3, Wire_10b (31)/3  "CYBER_FAULT"
  ASR903_2 (6)/2 -> Wire_5 (15)/2, Wire_9 (28)/2, Wire_3b (14)/2  "TLC_SERVICE"
  Wire_12 (38)/3 -> FG1500_1 (32)/3  "CYBER_FAULT"
  Wire_12 (38)/2 -> FG1500_1 (32)/2  "TLC_SERVICE"
  Wire_5b (16)/4 -> Wire_5 (15)/4  "MECH_FAULT"
  ASR920_1 (7)/3 -> Wire_6b (18)/3, Wire_12 (38)/3, Wire_14 (42)/3, Wire_15 (44)/3  "CYBER_FAULT"
  FG1500_1 (32)/1 -> Wire_12b (39)/1  "TLC_CONN"
  Wire_14 (42)/3 -> BIGP_1 (34)/3  "CYBER_FAULT"
  Wire_6b (18)/4 -> Wire_6 (17)/4  "MECH_FAULT"
  Wire_14 (42)/2 -> BIGP_1 (34)/2  "TLC_SERVICE"
  FG1500_1 (32)/3 -> Wire_12b (39)/3  "CYBER_FAULT"
  ASR920_2 (8)/2 -> Wire_5b (16)/2, Wire_18 (190)/2, Wire_17b (188)/2, Wire_11b (37)/2  "TLC_SERVICE"
  Wire_14 (42)/1 -> BIGP_1 (34)/1  "TLC_CONN"
  Wire_12 (38)/1 -> FG1500_1 (32)/1  "TLC_CONN"
  ASR9006_2 (10)/3 -> Wire_3 (11)/3, Wire_7 (19)/3, Wire_2b (97)/3  "CYBER_FAULT"
  FG1500_1 (32)/2 -> Wire_12b (39)/2  "TLC_SERVICE"
  ASR903_1 (5)/1 -> Wire_10b (31)/1, Wire_6 (17)/1, Wire_4 (12)/1  "TLC_CONN"
  ASR920_2 (8)/4 -> [Routing_QoS_920_2]  "ROUTING_QoS"
  Alcatel_1 (26)/2 -> Wire_10 (30)/2, 5G_Core_1 (198)/2, Cloud_Roma (238)/2  "TLC_SERVICE"
  Wire_4b (13)/4 -> Wire_4 (12)/4  "MECH_FAULT"
  R_Wire_1 (98)/1 -> TLC_conn1/1  "TLC_CONN"
  BIGP_1 (34)/2 -> Wire_14b (43)/2  "TLC_SERVICE"
  ROUTE_TIM_1 (20)/1 -> R_Wire_1 (98)/2  "TLC_SERVICE"
  ASR920_2 (8)/3 -> Wire_5b (16)/3, Wire_18 (190)/3, Wire_17b (188)/3, Wire_11b (37)/3  "CYBER_FAULT"
  R_Wire_1b (99)/4 -> R_Wire_1 (98)/4  "MECH_FAULT"
  R_Wire_1 (98)/4 -> R_Wire_1b (99)/4  "MECH_FAULT"
  Wire_10b (31)/4 -> Wire_10 (30)/4  "MECH_FAULT"
  Nex_1 (3)/4 -> [Switching_QoS_Nex_1]  "SWITCHING_QoS"
  Nex_2 (4)/4 -> [Switching_QoS_Nex_2]  "SWITCHING_QoS"
  Wire_1b (96)/4 -> Wire_1 (1)/4  "MECH_FAULT"
  Wire_1 (1)/4 -> Wire_1b (96)/4  "MECH_FAULT"
  Wire_2b (97)/4 -> Wire_2 (2)/4  "MECH_FAULT"
  Wire_2 (2)/4 -> Wire_2b (97)/4  "MECH_FAULT"
  Wire_15a (49)/4 -> Wire_15 (44)/4  "MECH_FAULT"
  Wire_15 (44)/4 -> Wire_15a (49)/4  "MECH_FAULT"
  CYBER_fault1/1 -> Nex_2 (4)/3  "CYBER_FAULT"
  TLC_conn3/1 -> ASR9006_2 (10)/1  "TLC_CONN"
  TLC_service3/1 -> ASR9006_2 (10)/2  "TLC_SERVICE"
  CYBER_fault3/1 -> ASR9006_2 (10)/3  "CYBER_FAULT"
  TLC_conn4/1 -> ASR9006_1 (9)/1  "TLC_CONN"
  TLC_service4/1 -> ASR9006_1 (9)/2  "TLC_SERVICE"
  CYBER_fault4/1 -> ASR9006_1 (9)/3  "CYBER_FAULT"
  TLC_conn5/1 -> ASR903_1 (5)/1  "TLC_CONN"
  TLC_service5/1 -> ASR903_1 (5)/2  "TLC_SERVICE"
  CYBER_fault5/1 -> ASR903_1 (5)/3  "CYBER_FAULT"
  TLC_conn6/1 -> ASR903_2 (6)/1  "TLC_CONN"
  TLC_service6/1 -> ASR903_2 (6)/2  "TLC_SERVICE"
  CYBER_fault6/1 -> ASR903_2 (6)/3  "CYBER_FAULT"
  TLC_conn8/1 -> ASR920_1 (7)/1  "TLC_CONN"
  TLC_service8/1 -> ASR920_1 (7)/2  "TLC_SERVICE"
  CYBER_fault8/1 -> ASR920_1 (7)/3  "CYBER_FAULT"
  Room_3 (200)/1 -> 5G_Core_1 (198)/5, Cloud_Roma (238)/5, Room_Qos12/2, Alcatel_1 (26)/5  "ROOM_QoS"
  Room_Qos12/1 -> Building_3 (215)/1  "ROOM_QoS"
  PowerGen_3 (157)/1 -> Alcatel_1 (26)/4, 5G_Core_1 (198)/4, Room_3 (200)/1, Cloud_Roma (238)/4, ASR903_1 (5)/4, Room_8 (283)/1  "POWER"
  TLC_conn9/1 -> Alcatel_1 (26)/1  "TLC_CONN"
  Cloud_Roma (238)/1 -> TLC_conn9/1  "TLC_CONN"
  Cloud_Roma (238)/2 -> TLC_service9/1  "TLC_SERVICE"
  Cloud_Roma (238)/3 -> CYBER_fault9/1  "CYBER_FAULT"
  Wire_10b (31)/1 -> TLC_conn9/2  "TLC_CONN"
  Wire_10b (31)/2 -> TLC_service9/2  "TLC_SERVICE"
  Wire_10b (31)/3 -> CYBER_fault9/2  "CYBER_FAULT"
  Wire_10 (30)/1 -> TLC_conn5/2  "TLC_CONN"
  Wire_10 (30)/2 -> TLC_service5/2  "TLC_SERVICE"
  Wire_10 (30)/3 -> CYBER_fault5/2  "CYBER_FAULT"
  Wire_4b (13)/1 -> TLC_conn5/1  "TLC_CONN"
  Wire_6b (18)/1 -> TLC_conn5/3  "TLC_CONN"
  Wire_6b (18)/2 -> TLC_service5/3  "TLC_SERVICE"
  Wire_4b (13)/2 -> TLC_service5/1  "TLC_SERVICE"
  Wire_4b (13)/3 -> CYBER_fault5/1  "CYBER_FAULT"
  Wire_6b (18)/3 -> CYBER_fault5/3  "CYBER_FAULT"
  Wire_8 (21)/1 -> TLC_conn4/1  "TLC_CONN"
  Wire_8 (21)/2 -> TLC_service4/1  "TLC_SERVICE"
  Wire_8 (21)/3 -> CYBER_fault4/1  "CYBER_FAULT"
  Wire_1 (1)/1 -> TLC_conn4/2  "TLC_CONN"
  Wire_1 (1)/2 -> TLC_service4/2  "TLC_SERVICE"
  Wire_1 (1)/3 -> CYBER_fault4/2  "CYBER_FAULT"
  Wire_4 (12)/1 -> TLC_conn4/3  "TLC_CONN"
  Wire_4 (12)/2 -> TLC_service4/3  "TLC_SERVICE"
  Wire_4 (12)/3 -> CYBER_fault4/3  "CYBER_FAULT"
  Wire_6 (17)/1 -> TLC_conn8/1  "TLC_CONN"
  Wire_6 (17)/2 -> TLC_service8/1  "TLC_SERVICE"
  Wire_6 (17)/3 -> CYBER_fault8/1  "CYBER_FAULT"
  Wire_12b (39)/1 -> TLC_conn8/2  "TLC_CONN"
  Wire_12b (39)/2 -> TLC_service8/2  "TLC_SERVICE"
  Wire_12b (39)/3 -> CYBER_fault8/2  "CYBER_FAULT"
  Wire_14b (43)/1 -> TLC_conn8/3  "TLC_CONN"
  Wire_14b (43)/2 -> TLC_service8/3  "TLC_SERVICE"
  Wire_14b (43)/3 -> CYBER_fault8/3  "CYBER_FAULT"
  Wire_15a (49)/1 -> TLC_conn8/4  "TLC_CONN"
  Wire_15a (49)/2 -> TLC_service8/4  "TLC_SERVICE"
  Wire_15a (49)/3 -> CYBER_fault8/4  "CYBER_FAULT"
  Room_1 (51)/1 -> Building_2 (201)/1, [Room_QoS_1]  "ROOM_QoS"
  PowerGen_1 (46)/1 -> [POWER_1], Room_1 (51)/1  "POWER"
  PowerGen_2 (47)/1 -> Room_2 (52)/1, [POWER_2]  "POWER"
  Room_2 (52)/1 -> [Room_QoS_2], Building_1 (53)/1  "ROOM_QoS"
  R_Wire_1b (99)/1 -> TLC_conn2/1  "TLC_CONN"
  R_Wire_1b (99)/2 -> TLC_service2/1  "TLC_SERVICE"
  R_Wire_1b (99)/3 -> CYBER_fault2/1  "CYBER_FAULT"
  Nex_2 (4)/1 -> Wire_7b (20)/1, Wire_1 (1)/1, R_Wire_1b (99)/1  "TLC_CONN"
  ROUTE_TIM_2 (21)/1 -> R_Wire_1b (99)/2  "TLC_SERVICE"
  Nex_2 (4)/3 -> Wire_7b (20)/3, Wire_1 (1)/3, R_Wire_1b (99)/3  "CYBER_FAULT"
  Wire_7b (20)/1 -> TLC_conn3/1  "TLC_CONN"
  Wire_7b (20)/2 -> TLC_service3/1  "TLC_SERVICE"
  Wire_7b (20)/3 -> CYBER_fault3/1  "CYBER_FAULT"
  Wire_2 (2)/1 -> TLC_conn3/2  "TLC_CONN"
  Wire_2 (2)/2 -> TLC_service3/2  "TLC_SERVICE"
  Wire_2 (2)/3 -> CYBER_fault3/2  "CYBER_FAULT"
  Wire_3b (14)/1 -> TLC_conn3/3  "TLC_CONN"
  Wire_3b (14)/2 -> TLC_service3/3  "TLC_SERVICE"
  Wire_3b (14)/3 -> CYBER_fault3/3  "CYBER_FAULT"
  ROUTE_TIM_1 (20)/2 -> Wire_8 (21)/2  "TLC_SERVICE"
  Nex_1 (3)/3 -> Wire_2 (2)/3, R_Wire_1 (98)/3, Wire_8 (21)/3  "CYBER_FAULT"
  ROUTE_TIM_1 (20)/3 -> Wire_2 (2)/2  "TLC_SERVICE"
  Wire_1b (96)/1 -> TLC_conn1/2  "TLC_CONN"
  ROUTE_TIM_2 (21)/2 -> Wire_1 (1)/2  "TLC_SERVICE"
  Wire_1b (96)/2 -> TLC_service1/2  "TLC_SERVICE"
  Wire_1b (96)/3 -> CYBER_fault1/2  "CYBER_FAULT"
  R_Wire_1 (98)/3 -> CYBER_fault1/1  "CYBER_FAULT"
  Wire_2b (97)/1 -> TLC_conn2/2  "TLC_CONN"
  Wire_2b (97)/2 -> TLC_service2/2  "TLC_SERVICE"
  Wire_2b (97)/3 -> CYBER_fault2/2  "CYBER_FAULT"
  Wire_8b (22)/1 -> TLC_conn2/3  "TLC_CONN"
  Wire_8b (22)/2 -> TLC_service2/3  "TLC_SERVICE"
  Wire_8b (22)/3 -> CYBER_fault2/3  "CYBER_FAULT"
  Wire_7 (19)/1 -> TLC_conn1/3  "TLC_CONN"
  Wire_7 (19)/2 -> TLC_service1/3  "TLC_SERVICE"
  Wire_7 (19)/3 -> CYBER_fault1/3  "CYBER_FAULT"
  Wire_3b (14)/4 -> Wire_3 (11)/4  "MECH_FAULT"
  Wire_3 (11)/1 -> TLC_conn6/1  "TLC_CONN"
  Wire_3 (11)/2 -> TLC_service6/1  "TLC_SERVICE"
  Wire_3 (11)/3 -> CYBER_fault6/1  "CYBER_FAULT"
  Wire_5b (16)/1 -> TLC_conn6/3  "TLC_CONN"
  Wire_5b (16)/2 -> TLC_service6/2  "TLC_SERVICE"
  Wire_5b (16)/3 -> CYBER_fault6/2  "CYBER_FAULT"
  Wire_9b (29)/1 -> TLC_conn6/2  "TLC_CONN"
  Wire_9b (29)/2 -> TLC_service6/3  "TLC_SERVICE"
  Wire_9b (29)/3 -> CYBER_fault6/3  "CYBER_FAULT"
  ROUTE_TIM_2 (21)/3 -> Wire_7b (20)/2  "TLC_SERVICE"
  Alcatel_2 (27)/1 -> Cloud_Milano (239)/1, Wire_9b (29)/1  "TLC_CONN"
  Cloud_Milano (239)/1 -> TLC_conn13/1  "TLC_CONN"
  Building5/1 -> Building_4 (216)/1  "ROOM_QoS"
  Cloud_Milano (239)/3 -> CYBER_fault10/1  "CYBER_FAULT"
  TLC_conn13/1 -> Alcatel_2 (27)/1  "TLC_CONN"
  Alcatel_2 (27)/3 -> Wire_9b (29)/3, Cloud_Milano (239)/3  "CYBER_FAULT"
  Cloud_Milano (239)/2 -> TLC_service10/1  "TLC_SERVICE"
  Alcatel_2 (27)/2 -> Wire_9b (29)/2, Cloud_Milano (239)/2  "TLC_SERVICE"
  Room_5 (240)/1 -> Alcatel_2 (27)/5, Cloud_Milano (239)/5, Building5/2  "ROOM_QoS"
  Wire_9 (28)/1 -> TLC_conn13/2  "TLC_CONN"
  Wire_9 (28)/2 -> TLC_service10/2  "TLC_SERVICE"
  Wire_9 (28)/3 -> CYBER_fault10/2  "CYBER_FAULT"
  Room_6 (241)/1 -> [Room_QoS]  "ROOM_QoS"
  PowerGen_6 (245)/1 -> [POWER], Room_6 (241)/1  "POWER"
  PowerGen_5 (236)/1 -> Cloud_Milano (239)/4, ASR903_2 (6)/4, Room_7 (252)/1, Room_5 (240)/1, Alcatel_2 (27)/4  "POWER"
  Room_7 (252)/1 -> ASR903_2 (6)/5, Building5/1  "ROOM_QoS"
  Room_8 (283)/1 -> ASR903_1 (5)/5, Room_Qos12/1  "ROOM_QoS"
  [POWER_4] -> Room_10 (257)/1, ASR920_1 (7)/4  "POWER"
  Room_10 (257)/1 -> ASR920_1 (7)/5  "ROOM_QoS"
  PowerGen_8 (281)/1 -> Room_4 (237)/1, ASR920_2 (8)/4, Room_9 (255)/1, BlockChainServer (256)/4, Alcatel_5 (292)/4  "POWER"
  Room_4 (237)/1 -> ASR920_2 (8)/5  "ROOM_QoS"
  Alcatel_2 (27)/4 -> [Routing_QoS_7750_2]  "ROUTING_QoS"
  Alcatel_5 (292)/4 -> [Routing_QoS_Alcatel_1]  "ROUTING_QoS"
  BlockChainServer (256)/1 -> TLC_conn10/1  "TLC_CONN"
  TLC_conn10/1 -> Alcatel_5 (292)/1  "TLC_CONN"
  BlockChainServer (256)/2 -> TLC_service12/1  "TLC_SERVICE"
  Room_9 (255)/1 -> BlockChainServer (256)/5, Alcatel_5 (292)/5  "ROOM_QoS"
  BlockChainServer (256)/3 -> CYBER_fault12/1  "CYBER_FAULT"
  TLC_conn11/1 -> ASR920_2 (8)/1  "TLC_CONN"
  TLC_service13/1 -> ASR920_2 (8)/2  "TLC_SERVICE"
  CYBER_fault13/1 -> ASR920_2 (8)/3  "CYBER_FAULT"
  Wire_5 (15)/1 -> TLC_conn11/1  "TLC_CONN"
  Wire_5 (15)/2 -> TLC_service13/1  "TLC_SERVICE"
  Wire_5 (15)/3 -> CYBER_fault13/1  "CYBER_FAULT"
  Alcatel_5 (292)/1 -> BlockChainServer (256)/1, Wire_11 (36)/1  "TLC_CONN"
  Alcatel_5 (292)/2 -> Wire_11 (36)/2, BlockChainServer (256)/2  "TLC_SERVICE"
  Alcatel_5 (292)/3 -> BlockChainServer (256)/3, Wire_11 (36)/3  "CYBER_FAULT"
  Wire_11 (36)/4 -> Wire_11b (37)/4  "MECH_FAULT"
  Wire_11 (36)/1 -> TLC_conn11/2  "TLC_CONN"
  Wire_11 (36)/2 -> TLC_service13/2  "TLC_SERVICE"
  Wire_11 (36)/3 -> CYBER_fault13/2  "CYBER_FAULT"
  Splitter_1 (54)/3 -> ONU_3 (282)/4  "NGPON_CONN"
  BLM_1500 (91)/3 -> Wire_15a (49)/3, Splitter_1 (54)/2  "CYBER_FAULT"
  [POWER_4] -> Room_12 (259)/1, ONU_3 (282)/3, BLM_1500 (91)/4  "POWER"
  Room_12 (259)/1 -> BLM_1500 (91)/5  "ROOM_QoS"
  BLM_1500 (91)/2 -> ROUTE_TIM_3 (22)/1  "TLC_SERVICE"
  BLM_1500 (91)/4 -> Splitter_1 (54)/3, [NGPON_CONN]  "NGPON_CONN"
  Splitter_1 (54)/2 -> ONU_3 (282)/2  "CYBER_FAULT"
  Splitter_1 (54)/1 -> ONU_3 (282)/1  "TLC_SERVICE"
  Splitter_1 (54)/4 -> BLM_1500 (91)/6  "NGPON_IN"
  Wire_15 (44)/1 -> BLM_1500 (91)/1  "TLC_CONN"
  Wire_15 (44)/2 -> BLM_1500 (91)/2  "TLC_SERVICE"
  Wire_15 (44)/3 -> BLM_1500 (91)/3  "CYBER_FAULT"
  BLM_1500 (91)/1 -> Wire_15a (49)/1  "TLC_CONN"
  ROUTE_TIM_3 (22)/1 -> Wire_15a (49)/2  "TLC_SERVICE"
  PowerGen_4 (214)/1 -> [POWER_4]  "POWER"
  ONU_3 (282)/3 -> Data Type Conversion/1  "NGPON_CONN"
  PowerGen_7 (260)/1 -> 5G_Pico_1 (192)/4, LocalCloud (261)/4, L2S_1 (226)/4, 5G_PGW_SGW_1 (193)/4, Room_14 (284)/1, RESISTO_1 (196)/4, Analytics_1 (195)/4, [POWER_7]  "POWER"
  Room_14 (284)/1 -> 5G_PGW_SGW_1 (193)/5, LocalCloud (261)/5, L2S_1 (226)/5  "ROOM_QoS"
  Data Type Conversion/1 -> L2S_1 (226)/1  "TLC_CONN"
  ONU_3 (282)/1 -> L2S_1 (226)/2  "TLC_SERVICE"
  5G_PGW_SGW_1 (193)/1 -> 5G_Pico_1 (192)/1  "TLC_CONN"
  5G_PGW_SGW_1 (193)/2 -> 5G_Pico_1 (192)/2, Display/1  "TLC_SERVICE"
  5G_PGW_SGW_1 (193)/3 -> 5G_Pico_1 (192)/3  "CYBER_FAULT"
  L2S_1 (226)/1 -> RESISTO_1 (196)/1, Analytics_1 (195)/1, LocalCloud (261)/1  "TLC_CONN"
  L2S_1 (226)/2 -> RESISTO_1 (196)/2, Analytics_1 (195)/2, LocalCloud (261)/2  "TLC_SERVICE"
  L2S_1 (226)/3 -> RESISTO_1 (196)/3, Analytics_1 (195)/3, LocalCloud (261)/3  "CYBER_FAULT"
  5G_Pico_1 (192)/2 -> Antenna_RU_2 (204)/2, Antenna_RU_1 (191)/2  "TLC_SERVICE"
  Analytics_1 (195)/1 -> WS/1  "WORKSTATION_QoS"
  RESISTO_1 (196)/1 -> WS/2  "WORKSTATION_QoS"
  Robot_1 (203)/1 -> ROBOT_QoS/1  "ROBOT_QoS"
  ROBOT_QoS/1 -> CELL_1 (271)/1  "ROBOT_QoS"
  Robot_2 (205)/1 -> ROBOT_QoS/2  "ROBOT_QoS"
  CELL_1 (271)/1 -> SAVE_18 (18)/1, [WORKING_CELL_QoS]  "WORKING_CELL_QoS"
  WS/1 -> SAVE_19 (19)/1  "WORKSTATION_QoS"
  Wire_MR_5 (139)/1 -> Medical_5 (175)/4  "POWER"
  Autoclave (121)/1 -> Pipe_Ward (127)/1  "WATER"
  Alcatel_4 (84)/3 -> Wire_18b (189)/3, Wire_19b (297)/3  "CYBER_FAULT"
  Wire_19 (296)/4 -> Wire_19b (297)/4  "MECH_FAULT"
  Duct_4 (170)/2 -> Mux3/3  "DUCT_QoS"
  Drug_Store (186)/1 -> Mux5/8  "ORDINARY_ROOM_QoS"
  Oxygen_Duct_2 (264)/1 -> Medical_2 (172)/8  "OXYGEN"
  Pipe_Medical5 (132)/1 -> Medical_5 (175)/5  "WATER"
  Staff_Room (183)/1 -> Mux5/6  "ORDINARY_ROOM_QoS"
  Oxygen_Duct_1 (263)/1 -> Medical_1 (171)/8  "OXYGEN"
  Pipe_Ward (127)/1 -> Pipe_Oper2 (135)/1, Pipe_Oper1 (134)/1, Pipe_Medical6 (133)/1, Pipe_Medical5 (132)/1, Pipe_Medical4 (131)/1, Pipe_Medical3 (130)/1, Pipe_Medical2 (129)/1, Pipe_Medical1 (128)/1  "WATER"
  Wire_18 (190)/1 -> TLC_conn15/1  "TLC_CONN"
  Mux5/1 -> media2/1(u)
  Tap (119)/1 -> Pipe_1 (120)/1  "WATER"
  Wire_17b (188)/3 -> CYBER_fault11/1  "CYBER_FAULT"
  [MOBILE_QoS] -> Medical_1 (171)/7, Medical_2 (172)/7, Medical_3 (173)/7, Medical_4 (174)/7, Medical_5 (175)/7, Medical_6 (176)/7, Operating_1 (177)/7, Operating_2 (178)/7  "MOBILE_QoS"
  Wire_17 (187)/4 -> Wire_17b (188)/4  "MECH_FAULT"
  Wire_OR_2 (164)/2 -> Mux1/3  "WIRE_QoS"
  Humidifier (124)/1 -> Cooling_Coil (125)/2  "AIR"
  Data_Room_1 (333)/1 -> L2S_2 (250)/5  "ROOM_QoS"
  Duct_2 (168)/1 -> Medical_3 (173)/6, Medical_4 (174)/6, Surgery (179)/2, Doctor_Room (115)/2, Waiting_Room (180)/2  "AIR"
  Wire_OP_1 (161)/1 -> Operating_1 (177)/4  "POWER"
  Pipe_Medical6 (133)/2 -> Mux4/6  "PIPE_QoS"
  Wire_18 (190)/4 -> Wire_18b (189)/4  "MECH_FAULT"
  Cooling_Coil (125)/1 -> Duct_4 (170)/1, Duct_3 (169)/1, Duct_2 (168)/1, Duct_1 (126)/1  "AIR"
  Pipe_Oper1 (134)/1 -> Operating_1 (177)/5  "WATER"
  BTS_1 (246)/3 -> ANT_1 (248)/4  "BTS_CONN"
  Pipe_Oper2 (135)/2 -> Mux4/8  "PIPE_QoS"
  Duct_3 (169)/2 -> Mux3/1  "DUCT_QoS"
  media/1(y) -> SAVE_16 (16)/1
  Wire_MR_3 (137)/2 -> Mux1/10  "WIRE_QoS"
  Pipe_Medical4 (131)/1 -> Medical_4 (174)/5  "WATER"
  Mux3/1 -> media/1(u)
  Wire_S_1 (166)/1 -> Oxygen_Pump (251)/1, Cooling_Coil (125)/1, Humidifier (124)/1, Heating_Coil (123)/1, Fan (122)/1  "POWER"
  [Room_QoS] -> Alcatel_3 (83)/5  "ROOM_QoS"
  Alcatel_3 (83)/4 -> [Routing_QoS_7750_3]  "ROUTING_QoS"
  TLC_conn15/1 -> Alcatel_4 (84)/1  "TLC_CONN"
  Medical_6 (176)/1 -> Mux7/6  "MEDICAL_ROOM_QoS"
  Pipe_Medical4 (131)/2 -> Mux4/4  "PIPE_QoS"
  Oxygen_Duct_6 (268)/1 -> Medical_6 (176)/8  "OXYGEN"
  Operating_2 (178)/1 -> Mux7/8  "MEDICAL_ROOM_QoS"
  Wire_19b (297)/2 -> MA5603 (95)/2  "TLC_SERVICE"
  Oxygen_Duct_5 (267)/1 -> Medical_5 (175)/8  "OXYGEN"
  Medical_4 (174)/1 -> Mux7/4  "MEDICAL_ROOM_QoS"
  Heating_Coil (123)/1 -> Humidifier (124)/2  "AIR"
  Duct_1 (126)/1 -> Operating_2 (178)/6, Operating_1 (177)/6  "AIR"
  Alcatel_4 (84)/4 -> [Routing_QoS_7750_4]  "ROUTING_QoS"
  Pipe_Medical2 (129)/2 -> Mux4/3  "PIPE_QoS"
  Wire_OR_1 (163)/2 -> Mux1/9  "WIRE_QoS"
  Alcatel_4 (84)/1 -> Wire_19b (297)/1, Wire_18b (189)/1  "TLC_CONN"
  Equipment_Warehouse (185)/1 -> Mux5/9  "ORDINARY_ROOM_QoS"
  Waiting_Room (180)/1 -> Mux5/3  "ORDINARY_ROOM_QoS"
  Wire_MR_3 (137)/1 -> Medical_3 (173)/4  "POWER"
  L2S_2 (250)/3 -> Medical_1 (171)/3, Operating_2 (178)/3, Operating_1 (177)/3, Medical_6 (176)/3, Medical_5 (175)/3, Medical_4 (174)/3, Medical_3 (173)/3, Medical_2 (172)/3  "CYBER_FAULT"
  Pipe_Oper1 (134)/2 -> Mux4/7  "PIPE_QoS"
  Wire_16a (50)/2 -> BTS_1 (246)/2  "TLC_SERVICE"
  Wire_S_1 (166)/2 -> Mux1/1  "WIRE_QoS"
  Wire_MR_4 (138)/2 -> Mux1/5  "WIRE_QoS"
  Pipe_Medical1 (128)/1 -> Medical_1 (171)/5  "WATER"
  MA5603 (95)/3 -> Wire_19 (296)/3, L2S_2 (250)/3  "CYBER_FAULT"
  Wire_MR_5 (139)/2 -> Mux1/4  "WIRE_QoS"
  Alcatel_3 (83)/3 -> Wire_16a (50)/3, Wire_17 (187)/3  "CYBER_FAULT"
  Fan (122)/1 -> Heating_Coil (123)/2  "AIR"
  TLC_service11/1 -> Alcatel_3 (83)/2  "TLC_SERVICE"
  media4/1(y) -> SAVE_13 (13)/1  "PIPE_QoS"
  Oxygen_Duct_4 (266)/1 -> Medical_4 (174)/8  "OXYGEN"
  Pipe_Medical2 (129)/1 -> Medical_2 (172)/5  "WATER"
  Wire_16a (50)/3 -> BTS_1 (246)/3  "CYBER_FAULT"
  BTS_1 (246)/2 -> Wire_16 (45)/3, ANT_1 (248)/2  "CYBER_FAULT"
  Alcatel_4 (84)/2 -> Wire_19b (297)/2, Wire_18b (189)/2  "TLC_SERVICE"
  Wire_16a (50)/4 -> Wire_16 (45)/4  "MECH_FAULT"
  Wire_19 (296)/3 -> CYBER_fault14/2  "CYBER_FAULT"
  CYBER_fault11/1 -> Alcatel_3 (83)/3  "CYBER_FAULT"
  Operating_1 (177)/1 -> Mux7/7  "MEDICAL_ROOM_QoS"
  media1/1(y) -> SAVE_17 (17)/1
  Wire_19b (297)/3 -> MA5603 (95)/3  "CYBER_FAULT"
  Wire_OP_1 (161)/2 -> Mux1/8  "WIRE_QoS"
  Pipe_Oper2 (135)/1 -> Operating_2 (178)/5  "WATER"
  Wire_16 (45)/1 -> TLC_conn14/2  "TLC_CONN"
  Mobile_1 (147)/1 -> SAVE_9 (9)/1, [MOBILE_QoS]  "MOBILE_QoS"
  Wire_17b (188)/2 -> TLC_service11/1  "TLC_SERVICE"
  Medical_5 (175)/1 -> Mux7/5  "MEDICAL_ROOM_QoS"
  Mux1/1 -> media1/1(u)
  Mux7/1 -> media3/1(u)
  Wire_16a (50)/1 -> BTS_1 (246)/1  "TLC_CONN"
  BTS_1 (246)/1 -> ANT_1 (248)/1, Wire_16 (45)/2  "TLC_SERVICE"
  MA5603 (95)/4 -> [ADSL_QoS]  "ADSL_CONN"
  TLC_conn14/1 -> Alcatel_3 (83)/1  "TLC_CONN"
  Pipe_Medical6 (133)/1 -> Medical_6 (176)/5  "WATER"
  Wire_16 (45)/4 -> Wire_16a (50)/4  "MECH_FAULT"
  Pipe_Medical3 (130)/1 -> Medical_3 (173)/5  "WATER"
  [POWER] -> Alcatel_4 (84)/4  "POWER"
  Oxygen_Duct_8 (270)/1 -> Operating_2 (178)/8  "OXYGEN"
  Wire_19 (296)/2 -> TLC_service14/2  "TLC_SERVICE"
  Wire_OR_3 (165)/2 -> Mux1/2  "WIRE_QoS"
  Pipe_1 (120)/2 -> Mux4/9  "PIPE_QoS"
  media2/1(y) -> SAVE_14 (14)/1  "ORDINARY_ROOM_QoS"
  Wire_18 (190)/2 -> TLC_service14/1  "TLC_SERVICE"
  Medical_1 (171)/1 -> Mux7/1  "MEDICAL_ROOM_QoS"
  Duct_1 (126)/2 -> Mux3/4  "DUCT_QoS"
  MA5603 (95)/1 -> L2S_2 (250)/1, Wire_19 (296)/1  "TLC_CONN"
  Wire_19b (297)/1 -> MA5603 (95)/1  "TLC_CONN"
  Wire_18 (190)/3 -> CYBER_fault14/1  "CYBER_FAULT"
  CYBER_fault14/1 -> Alcatel_4 (84)/3  "CYBER_FAULT"
  [POWER] -> MA5603 (95)/4  "POWER"
  Wire_18b (189)/4 -> Wire_18 (190)/4  "MECH_FAULT"
  Oxygen_Duct_3 (265)/1 -> Medical_3 (173)/8  "OXYGEN"
  Cafeteria (181)/1 -> Mux5/4  "ORDINARY_ROOM_QoS"
  Medical_2 (172)/1 -> Mux7/2  "MEDICAL_ROOM_QoS"
  Oxygen_Duct_7 (269)/1 -> Operating_1 (177)/8  "OXYGEN"
  [Room_QoS] -> Alcatel_4 (84)/5  "ROOM_QoS"
  Medical_3 (173)/1 -> Mux7/3  "MEDICAL_ROOM_QoS"
  Visit_Room (184)/1 -> Mux5/7  "ORDINARY_ROOM_QoS"
  Wire_MR_1 (118)/2 -> Mux1/12  "WIRE_QoS"
  L2S_2 (250)/1 -> Display10/1, Display9/1, Medical_1 (171)/1, Operating_2 (178)/1, Operating_1 (177)/1, Medical_6 (176)/1, Medical_5 (175)/1, Medical_4 (174)/1, Medical_3 (173)/1, Medical_2 (172)/1  "TLC_CONN"
  Wire_19 (296)/1 -> TLC_conn15/2  "TLC_CONN"
  Doctor_Room (115)/1 -> Mux5/1  "ORDINARY_ROOM_QoS"
  Generator (116)/1 -> Wire_S_1 (166)/1, Wire_OP_2 (162)/1, Wire_OP_1 (161)/1, Wire_MR_6 (140)/1, Wire_MR_5 (139)/1, Wire_MR_4 (138)/1, Wire_MR_3 (137)/1, Wire_MR_2 (136)/1, Wire_S_2 (167)/1, L2S_2 (250)/4, Wire_MR_1 (118)/1, Data_Room_1 (333)/1, Wire_OR_3 (165)/1, Wire_OR_2 (164)/1, Wire_OR_1 (163)/1  "POWER"
  Surgery (179)/1 -> Mux5/2  "ORDINARY_ROOM_QoS"
  Alcatel_3 (83)/1 -> Wire_17 (187)/1, Wire_16a (50)/1, Wire_16 (45)/1  "TLC_CONN"
  Pipe_1 (120)/1 -> Autoclave (121)/2  "WATER"
  Wire_MR_4 (138)/1 -> Medical_4 (174)/4  "POWER"
  Wire_16 (45)/2 -> TLC_service11/2  "TLC_SERVICE"
  Duct_2 (168)/2 -> Mux3/2  "DUCT_QoS"
  Wire_OR_2 (164)/1 -> Cafeteria (181)/1, Material_Room (182)/1, Staff_Room (183)/1, Visit_Room (184)/1  "POWER"
  Wire_19b (297)/4 -> Wire_19 (296)/4  "MECH_FAULT"
  Pipe_Medical3 (130)/2 -> Mux4/2  "PIPE_QoS"
  L2S_2 (250)/2 -> Display19/1, Medical_1 (171)/2, Operating_2 (178)/2, Operating_1 (177)/2, Medical_6 (176)/2, Medical_5 (175)/2, Medical_4 (174)/2, Medical_3 (173)/2, Medical_2 (172)/2  "TLC_SERVICE"
  Wire_OP_2 (162)/1 -> Operating_2 (178)/4  "POWER"
  Alcatel_3 (83)/2 -> Wire_16a (50)/2, Wire_17 (187)/2  "TLC_SERVICE"
  PowerGen_9 (294)/1 -> ANT_1 (248)/3  "POWER"
  Material_Room (182)/1 -> Mux5/5  "ORDINARY_ROOM_QoS"
  Oxygen_Pump (251)/1 -> Oxygen_Duct_7 (269)/1, Oxygen_Duct_8 (270)/1, Oxygen_Duct_6 (268)/1, Oxygen_Duct_5 (267)/1, Oxygen_Duct_4 (266)/1, Oxygen_Duct_3 (265)/1, Oxygen_Duct_2 (264)/1, Oxygen_Duct_1 (263)/1  "OXYGEN"
  Wire_OR_1 (163)/1 -> Waiting_Room (180)/1, Surgery (179)/1, Doctor_Room (115)/1  "POWER"
  Duct_4 (170)/1 -> Medical_6 (176)/6, Medical_5 (175)/6, Equipment_Warehouse (185)/2, Drug_Store (186)/2  "AIR"
  Wire_MR_2 (136)/1 -> Medical_2 (172)/4  "POWER"
  Mux4/1 -> media4/1(u)
  Wire_MR_6 (140)/1 -> Medical_6 (176)/4  "POWER"
  media3/1(y) -> SAVE_15 (15)/1, [MEDICAL_ROOM_QoS]  "MEDICAL_ROOM_QoS"
  Pipe_Medical5 (132)/2 -> Mux4/5  "PIPE_QoS"
  Wire_MR_6 (140)/2 -> Mux1/6  "WIRE_QoS"
  Pipe_Medical1 (128)/2 -> Mux4/1  "PIPE_QoS"
  Wire_OR_3 (165)/1 -> Drug_Store (186)/1, Equipment_Warehouse (185)/1  "POWER"
  TLC_service14/1 -> Alcatel_4 (84)/2  "TLC_SERVICE"
  Pipe_Ward (127)/2 -> Mux4/10  "PIPE_QoS"
  Wire_OP_2 (162)/2 -> Mux1/7  "WIRE_QoS"
  Wire_MR_2 (136)/2 -> Mux1/11  "WIRE_QoS"
  [POWER] -> Alcatel_3 (83)/4  "POWER"
  Wire_16 (45)/3 -> CYBER_fault11/2  "CYBER_FAULT"
  Duct_3 (169)/1 -> Medical_1 (171)/6, Medical_2 (172)/6, Staff_Room (183)/2, Visit_Room (184)/2, Cafeteria (181)/2, Material_Room (182)/2  "AIR"
  Wire_17b (188)/4 -> Wire_17 (187)/4  "MECH_FAULT"
  Wire_17b (188)/1 -> TLC_conn14/1  "TLC_CONN"
  Wire_11b (37)/4 -> Wire_11 (36)/4  "MECH_FAULT"
  Wire_11b (37)/1 -> TLC_conn10/2  "TLC_CONN"
  Wire_11b (37)/2 -> TLC_service12/2  "TLC_SERVICE"
  Wire_11b (37)/3 -> CYBER_fault12/2  "CYBER_FAULT"
  TLC_service9/1 -> Alcatel_1 (26)/2  "TLC_SERVICE"
  CYBER_fault9/1 -> Alcatel_1 (26)/3  "CYBER_FAULT"
  TLC_service10/1 -> Alcatel_2 (27)/2  "TLC_SERVICE"
  CYBER_fault10/1 -> Alcatel_2 (27)/3  "CYBER_FAULT"
  TLC_service12/1 -> Alcatel_5 (292)/2  "TLC_SERVICE"
  CYBER_fault12/1 -> Alcatel_5 (292)/3  "CYBER_FAULT"
  ROUTE_TIM_3 (22)/2 -> Splitter_1 (54)/1  "TLC_SERVICE"
  PowerGen_10 (293)/1 -> [POWER_10], Room_13 (262)/1, Robot_1 (203)/2, Robot_2 (205)/2, Antenna_RU_1 (191)/4, Antenna_RU_2 (204)/4  "POWER"
  Alcatel_1 (26)/4 -> [Routing_QoS_7750_1]  "ROUTING_QoS"
  Room_13 (262)/1 -> 5G_Pico_1 (192)/5  "ROOM_QoS"
  5G_Core_1 (198)/1 -> TLC_conn9/3  "TLC_CONN"
  5G_Core_1 (198)/2 -> TLC_service9/3  "TLC_SERVICE"
  5G_Core_1 (198)/3 -> CYBER_fault9/3  "CYBER_FAULT"
  MA5603 (95)/2 -> ROUTE_TIM_4 (23)/1  "TLC_SERVICE"
  ROUTE_TIM_4 (23)/2 -> L2S_2 (250)/2  "TLC_SERVICE"
  ROUTE_TIM_4 (23)/1 -> Wire_19 (296)/2  "TLC_SERVICE"
  Alcatel_1 (26)/3 -> 5G_Core_1 (198)/3, Cloud_Roma (238)/3, Wire_10 (30)/3  "CYBER_FAULT"
  5G_Pico_1 (192)/1 -> Antenna_RU_2 (204)/1, Antenna_RU_1 (191)/1  "TLC_CONN"
  5G_Pico_1 (192)/3 -> Antenna_RU_2 (204)/3, Antenna_RU_1 (191)/3  "CYBER_FAULT"
  ASR9006_1 (9)/3 -> Wire_8b (22)/3, Wire_1b (96)/3, Wire_4b (13)/3  "CYBER_FAULT"
  5G_Core_1 (198)/4 -> Demux/1  "STATE"
  Demux/1 -> Terminator/1
  ONU_3 (282)/2 -> L2S_1 (226)/3  "CYBER_FAULT"
  LocalCloud (261)/1 -> 5G_PGW_SGW_1 (193)/1  "TLC_CONN"
  LocalCloud (261)/2 -> 5G_PGW_SGW_1 (193)/2  "TLC_SERVICE"
  LocalCloud (261)/3 -> 5G_PGW_SGW_1 (193)/3  "CYBER_FAULT"
  BlockChainServer (256)/4 -> Demux4/1  "STATE"
  Demux4/1 -> Terminator5/1
  ANT_1 (248)/1 -> Display6/1, Mobile_1 (147)/1  "TLC_SERVICE"
  ANT_1 (248)/2 -> Mobile_1 (147)/2  "CYBER_FAULT"
  ANT_1 (248)/3 -> Display7/1, Mobile_1 (147)/3  "R_CONN"
  Antenna_RU_1 (191)/3 -> Display8/1, Robot_1 (203)/3  "R_CONN"
  Antenna_RU_2 (204)/3 -> Robot_2 (205)/3  "R_CONN"
  Wire_18b (189)/1 -> TLC_conn11/3  "TLC_CONN"
  Wire_18b (189)/2 -> TLC_service13/3  "TLC_SERVICE"
  Wire_18b (189)/3 -> CYBER_fault13/3  "CYBER_FAULT"
  Wire_17 (187)/1 -> TLC_conn11/4  "TLC_CONN"
  Wire_17 (187)/2 -> TLC_service13/4  "TLC_SERVICE"
  Wire_17 (187)/3 -> CYBER_fault13/4  "CYBER_FAULT"
  Antenna_RU_1 (191)/1 -> Robot_1 (203)/1  "TLC_SERVICE"
  Antenna_RU_2 (204)/1 -> Robot_2 (205)/1  "TLC_SERVICE"
  Building_1 (53)/2 -> [Building_QoS_1]  "BUILDING_QoS"
  [Robot_Alt_Rout_2] -> Mux10/4
  media13/1(y) -> SAVE_23 (23)/1  "ALT_PORT_ISOLATION"
  [Routing_QoS_903_2] -> Mux2/8
  media6/1(y) -> SAVE_5 (5)/1, Subsystem12/2(2)  "ROUTING_QoS"
  [Medical_Alt_Serv_1] -> Mux9/2
  Mux2/1 -> media6/1(u), Display5/1
  [Routing_QoS_9006_2] -> Mux2/6
  [FW_QoS_1] -> SAVE_1 (1)/1  "FIREWALL_GLOBAL_QoS"
  Subsystem12/1(MEAN) -> SAVE_4 (4)/1, Mux8/2  "MPLS_NET_QoS"
  media5/1(y) -> SAVE_8 (8)/1  "GLOBAL_QoS"
  [Robot_Alt_Rout_1] -> Mux10/3
  [MEDICAL_ROOM_QoS] -> Mux6/2
  Constant5/1 -> SAVE_7 (7)/1, Mux8/1  "REDUNDANCY_QoS"
  [Routing_QoS_9006_1] -> Mux2/5
  [Routing_QoS_Alcatel_1] -> Mux2/11
  media8/1(y) -> SAVE_6 (6)/1, Subsystem12/1(1)  "SWITCHING_QoS"
  Max/1 -> media10/1(u)
  [Routing_QoS_7750_1] -> Mux2/1
  media12/1(y) -> SAVE_3 (3)/1  "BUILDING_QoS"
  Mux8/1 -> media5/1(u)
  [Robot_Alt_Serv_2] -> Mux9/4
  [Robot_Alt_Serv_1] -> Mux9/3
  Mux9/1 -> Display16/1, media9/1(u), Max/2
  media7/1(y) -> SAVE_2 (2)/1, Mux8/3  "SERVICES_QoS"
  media9/1(y) -> SAVE_21 (21)/1  "ALT_SERVICES"
  [Mobile_Alt_Serv_1] -> Mux9/1
  [Routing_QoS_7750_2] -> Mux2/2
  [Routing_QoS_920_2] -> Mux2/10
  Constant/1 -> Max/3, media13/1(u)
  [MOBILE_QoS] -> Mux6/1
  Mux13/1 -> media8/1(u)
  [Routing_QoS_920_1] -> Mux2/9
  [Routing_QoS_7750_4] -> Mux2/4
  [Mobile_Alt_Rout_1] -> Mux10/1
  Mux10/1 -> Display15/1, Max/1, media11/1(u)
  media10/1(y) -> SAVE_22 (22)/1  "ALT_ALL"
  Mux6/1 -> media7/1(u), Display22/1
  [WORKING_CELL_QoS] -> Mux6/3
  [Medical_Alt_Rout_1] -> Mux10/2
  [Routing_QoS_7750_3] -> Mux2/3
  media11/1(y) -> SAVE_20 (20)/1  "ALT_ROUTING"
  [Routing_QoS_903_1] -> Mux2/7
  Building_4 (216)/2 -> [Building_QoS_4]  "BUILDING_QoS"
  Building_2 (201)/2 -> [Building_QoS_2]  "BUILDING_QoS"
  Building_3 (215)/2 -> [Building_QoS_3]  "BUILDING_QoS"
  Mux12/1 -> media12/1(u)
  [Building_QoS_1] -> Mux12/1
  [Building_QoS_4] -> Mux12/4
  [Building_QoS_3] -> Mux12/3
  [Building_QoS_2] -> Mux12/2
  [Switching_QoS_Nex_1] -> Mux13/1
  [Switching_QoS_Nex_2] -> Mux13/2
  Mobile_1 (147)/4 -> [Mobile_Alt_Port_1]  "ALT_PORT_ISOLATION"
  Mobile_1 (147)/3 -> [Mobile_Alt_Serv_1]  "ALT_SERVICES"
  Mobile_1 (147)/2 -> [Mobile_Alt_Rout_1]  "ALT_ROUTING"
  Medical_1 (171)/2 -> [Medical_Alt_Rout_1]  "ALT_ROUTING"
  Medical_1 (171)/3 -> [Medical_Alt_Serv_1]  "ALT_SERVICES"
  Robot_1 (203)/2 -> [Robot_Alt_Rout_1]  "ALT_ROUTING"
  Robot_1 (203)/3 -> [Robot_Alt_Serv_1]  "ALT_SERVICES"
  Robot_2 (205)/2 -> [Robot_Alt_Rout_2]  "ALT_ROUTING"
  Robot_2 (205)/3 -> [Robot_Alt_Serv_2]  "ALT_SERVICES"
  CISIA_MASTER (0)/4 -> Display21/1  "TIME PAST"
  CISIA_MASTER (0)/2 -> Display11/1  "MAJOR HITS"
  CISIA_MASTER (0)/3 -> Display20/1  "DELTA TIME"
  CISIA_MASTER (0)/1 -> Display18/1  "MINOR HITS"
  Wire_MR_1 (118)/1 -> Medical_1 (171)/4  "POWER"
  Wire_S_2 (167)/1 -> Autoclave (121)/1  "POWER"
  Wire_S_2 (167)/2 -> Mux1/13  "WIRE_QoS"
